simulink model "HIL_Testing_SW_amantest"  (Simulink 7.5)
settings: Solver=ode1  StartTime=0.0  StopTime=Inf  FixedStep=0.001  RelTol=1e-3
PostLoadFcn:
  | , if any(exist('dsrtsu_mdlpostloadfcn', 'file') == [2, 3, 6]), try dsrtsu_mdlpostloadfcn('Execute', bdroot); catch fprintf('Error in PostLoadFcn (dsrtsu_mdlpostloadfcn) for model "%s":\n %s\n', bdroot, lasterr); end, end,
undefined symbols (not defined in the file): CeBSER_Cnt_NumTempAxisPts, ChargeCord, ChargeCord_Control, ChargeToSOCCurr, ChrgCurrLim, CrntSens1Fine, CS_SOCSetPt, CyclerMaxChrgPwr, CyclerMaxDschrgPwr, deltaAhr, Drive_1, Drive_10, Drive_11, Drive_12, Drive_13, Drive_14, Drive_15, Drive_16, Drive_17, Drive_18, Drive_19, Drive_2, Drive_20, Drive_21, Drive_22, Drive_23, Drive_24, Drive_25, Drive_26, Drive_27, Drive_28, Drive_29, Drive_3, Drive_30, Drive_31, Drive_32, Drive_33, Drive_34, Drive_35, Drive_36, Drive_37, Drive_38, Drive_39, Drive_4, Drive_40, Drive_41, Drive_42, Drive_43, Drive_44, Drive_45, Drive_46, Drive_47, Drive_48, Drive_49, Drive_5, Drive_50, Drive_51, Drive_6, Drive_7, Drive_8 ... (+50)
libraries: simulink x129, rtican x50, rti2211sailib x5, rti2211serlib x5, rti2202miolib x3
(part 14 of 23)

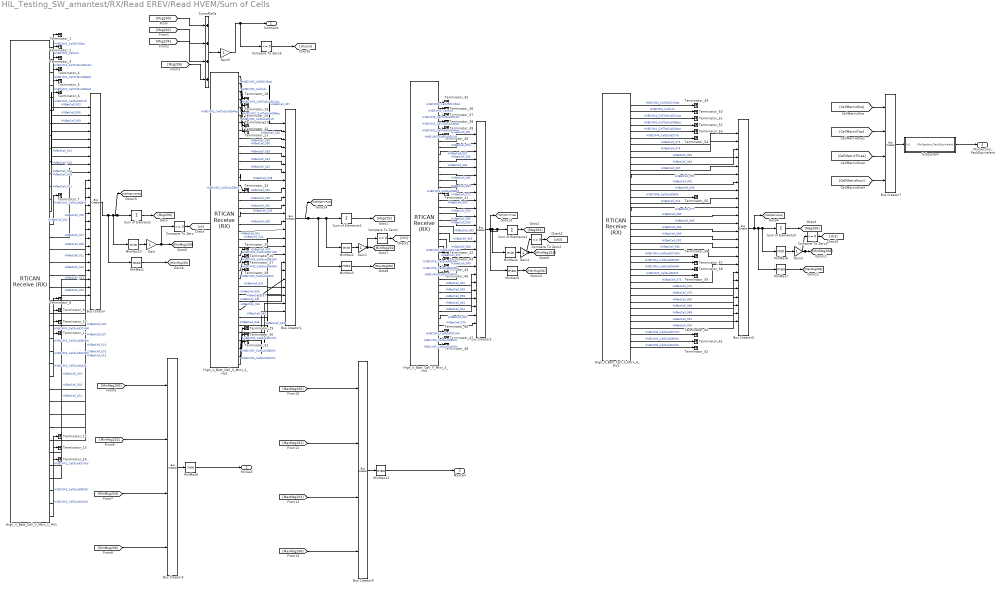
== system HIL_Testing_SW_amantest/RX/Read EREV/Read HVEM/Sum of Cells ==
  Bus Creator{,1..3} (4 alike) : BusCreator  Inputs=24
  Bus Creator5 : BusCreator
  Bus Creator6 : BusCreator
  Bus Creator7 : BusCreator
  Compare To Zero{,1..3,5} (5 alike) : simulink/Logic and Bit Operations/Compare To Zero  SystemSampleTime=-1  relop=<=  LogicOutDataTypeMode=uint8  ZeroCross=off
  Gain{,1..3,5} (5 alike) : Gain  ParameterDataType=sfix(16)  ParameterScaling=2^0  OutDataType=sfix(16)  OutScaling=2^0
  High_V_Batt_Cell_V_Mtrx_1_HV1 : rtican/RTICAN Receive (RX)   SystemSampleTime=-1  Reserved1=[]  Reserved2=[]  Reserved3=[]  Reserved4=[]  SfcnMessage=[]  Msg_Struct=[]  BoardTypeNo=[]  BoardNo=[]  ChannelNo=[]  Parameters=[]  DialogFcn=[]  UnitName=[]  Revision=[]  UnitValues=[]  DSProperties=struct('RTI',struct('Version',uint32(5),'BlockType',struct('isSLSource',uint8(1),'isSLSink',uint8(1),'isHWSource',uint8(0),'isHWSink',uint8(0),'isSetup',uint8(0),'isInline',uint8(1),'isNonInline',uint8(0),'isInterrupt',uint8(0),'isChannelwise',uint8(0)),'IOBoardType','RTICAN','UnitType','MESSAGE','Identifier','RX','DialogType','MSVC','BlockSet','RTICAN','SlaveProcessor','CAN'))  RTIBlockInterface=struct('OutputPortsWidth',int32([1 1 1 1 1 1 1 1 1 1 1 1 1 1 1 1 1 1 1 1 1 1 1 1 1 1 1 1 1 1 1 1 1 1 1 1 1 1]),'OutputPortsActive',[1 1 1 1 1 1 1 1 1 1 1 1 1 1 1 1 1 1 1 1 1 1 1 1 1 1 1 1 1 1 1 1 1 1 1 1 1 1],'OutputPortsName',{{'HVBCVM1_CellOCVStat','HVBCVM1_CellIndx','HVBCVM1_CellTstSubIDCAct','HVBCVM1_CellTstSubIDBAct','HVBCVM1_CellTstSubIDAAct','HVBCVM1_CellSubIDCVlt','HVBatCell_003','HVBatCell_006','HVBatCell_009','HVBatCell_012','HVBatCell_015','HVBatCell_018','HVBatCell_021','HVBatCell_024','HVBCVM1_CellSubIDBVlt','HVBatCell_002','HVBatCell_005','HVBatCell_008','HVBatCell_011','HVBatCell_014','HVBatCell_017','HVBatCell_020','HVBatCell_023','HVBCVM1_CellSubIDCVltM','HVBCVM1_CellSubIDBVltM','HVBCVM1_CellSubIDAVltM','HVBCVM1_CellSubIDAVlt','HVBatCell_001','HVBatCell_004','HVBatCell_007','HVBatCell_010','HVBatCell_013','HVBatCell_016','HVBatCell_019','HVBatCell_022','HVBCVM1_CellSubIDCVltV','HVBCVM1_CellSubIDBVltV','HVBCVM1_CellSubIDAVltV'}},'OutputPortsDataType',{{'SS_DOUBLE','SS_DOUBLE','SS_DOUBLE','SS_DOUBLE','SS_DOUBLE','SS_DOUBLE','SS_DOUBLE','SS_DOUBLE','SS_DOUBLE','SS_DOUBLE','SS_DOUBLE','SS_DOUBLE','SS_DOUBLE','SS_DOUBLE','SS_DOUBLE','SS_DOUBLE','SS_DOUBLE','SS_DOUBLE','SS_DOUBLE','SS_DOUBLE','SS_DOUBLE','SS_DOUBLE','SS_DOUBLE','SS_DOUBLE','SS_DOUBLE','SS_DOUBLE','SS_DOUBLE','SS_DOUBLE','SS_DOUBLE','SS_DOUBLE','SS_DOUBLE','SS_DOUBLE','SS_DOUBLE','SS_DOUBLE','SS_DOUBLE','SS_DOUBLE','SS_DOUBLE','SS_DOUBLE'}},'OutputPortsLabel',{{'HVBCVM1_CellOCVStat','HVBCVM1_CellIndx','HVBCVM1_CellTstSubIDCAct','HVBCVM1_CellTstSubIDBAct','HVBCVM1_CellTstSubIDAAct','HVBCVM1_CellSubIDCVlt','HVBatCell_003','HVBatCell_006','HVBatCell_009','HVBatCell_012','HVBatCell_015','HVBatCell_018','HVBatCell_021','HVBatCell_024','HVBCVM1_CellSubIDBVlt','HVBatCell_002','HVBatCell_005','HVBatCell_008','HVBatCell_011','HVBatCell_014','HVBatCell_017','HVBatCell_020','HVBatCell_023','HVBCVM1_CellSubIDCVltM','HVBCVM1_CellSubIDBVltM','HVBCVM1_CellSubIDAVltM','HVBCVM1_CellSubIDAVlt','HVBatCell_001','HVBatCell_004','HVBatCell_007','HVBatCell_010','HVBatCell_013','HVBatCell_016','HVBatCell_019','HVBatCell_022','HVBCVM1_CellSubIDCVltV','HVBCVM1_CellSubIDBVltV','HVBCVM1_CellSubIDAVltV'}},'OutputPortsLabelMode','ON','InputPortsWidth',int32(0),'InputPortsActive',0,'DialogFcn','rtican_message_interface_gui','BlockDisplay',{{'','center'}},'IconTransparency','on','ParameterTunableNames',{{}},'InitLevel',3,'BlockName',struct('Token',{{'High_V_Batt_Cell_V_Mtrx_1_HV'}}),'SampleTime',{{-1}},'TriggerPort',{{'none'}},'EnablePort',{{'none'}})  RTIBlockParameters=struct('BoardTypeNo',{{4302,'OFF',[]}},'BoardNo',{{1,'ON',[1 16]}},'ChannelNo',{{4,'ON',[1 4]}},'Parameters',{{struct('DataFileSupport',struct('DataFileSelectedMaster',1,'DataFileSelectedLocal',1,'DataFileName',['c:\data\databases\8.0.0 (12505)\globala - hv.dbc|c:\data\testing\dbc\globala - hvdmx112.dbc|'],'DataFileDate',{{{['06-Jan-2012 10:17:38']},{['10-May-2011 15:46:00']}}},'SelectedFile',['dbc\globala - hvdmx112.dbc']),'Options',struct('StatusSelected',0,'TimeSelected',0,'DeltaTimeSelected',0,'BytePortSelected',0,'MessageLengthSelected',0,'TriggerPort',struct('Selected',0,'TriggerType',0),'UserCoding',struct('Selected',0,'InterfaceFile','UserDecodingFile','FcnName','UserDecodeFcn','InportSelected',0,'InportWidth',1,'OutportSelected',0,'OutportWidth',1),'EnablePortSelected',0,'SignalOnPortnameSelected',1,'UseRXService',0),'Message',struct('MsgOnBlocknameSelected',1,'MsgName','High_V_Batt_Cell_V_Mtrx_1_HV','MsgIdFormat',0,'MsgId',512,'MsgLength',8,'NumSignals',38,'SampleTime',-1,'Signal',struct('SgnName',{'HVBCVM1_CellOCVStat','HVBCVM1_CellIndx','HVBCVM1_CellTstSubIDCAct','HVBCVM1_CellTstSubIDBAct','HVBCVM1_CellTstSubIDAAct','HVBCVM1_CellSubIDCVlt','HVBatCell_003','HVBatCell_006','HVBatCell_009','HVBatCell_012','HVBatCell_015','HVBatCell_018','HVBatCell_021','HVBatCell_024','HVBCVM1_CellSubIDBVlt','HVBatCell_002','HVBatCell_005','HVBatCell_008','HVBatCell_011','HVBatCell_014','HVBatCell_017','HVBatCell_020','HVBatCell_023','HVBCVM1_CellSubIDCVltM','HVBCVM1_CellSubIDBVltM','HVBCVM1_CellSubIDAVltM','HVBCVM1_CellSubIDAVlt','HVBatCell_001','HVBatCell_004','HVBatCell_007','HVBatCell_010','HVBatCell_013','HVBatCell_016','HVBatCell_019','HVBatCell_022','HVBCVM1_CellSubIDCVltV','HVBCVM1_CellSubIDBVltV','HVBCVM1_CellSubIDAVltV'},'SgnStartBit',{11,12,16,17,18,19,19,19,19,19,19,19,19,19,32,32,32,32,32,32,32,32,32,45,46,47,48,48,48,48,48,48,48,48,48,61,62,63},'SgnLength',{1,4,1,1,1,13,13,13,13,13,13,13,13,13,13,13,13,13,13,13,13,13,13,1,1,1,13,13,13,13,13,13,13,13,13,1,1,1},'SgnType',{0,1,0,0,0,0,2,2,2,2,2,2,2,2,0,2,2,2,2,2,2,2,2,0,0,0,0,2,2,2,2,2,2,2,2,0,0,0},'ModeValue',{-1,-1,-1,-1,-1,-1,1,3,5,7,9,11,13,15,-1,1,3,5,7,9,11,13,15,-1,-1,-1,-1,1,3,5,7,9,11,13,15,-1,-1,-1},'DataType',{0,0,0,0,0,0,0,0,0,0,0,0,0,0,0,0,0,0,0,0,0,0,0,0,0,0,0,0,0,0,0,0,0,0,0,0,0,0},'ByteLayout',{2,2,2,2,2,2,2,2,2,2,2,2,2,2,2,2,2,2,2,2,2,2,2,2,2,2,2,2,2,2,2,2,2,2,2,2,2,2},'Factor',{1,1,1,1,1,0.000625,0.000625,0.000625,0.000625,0.000625,0.000625,0.000625,0.000625,0.000625,0.000625,0.000625,0.000625,0.000625,0.000625,0.000625,0.000625,0.000625,0.000625,1,1,1,0.000625,0.000625,0.000625,0.000625,0.000625,0.000625,0.000625,0.000625,0.000625,1,1,1},'Offset',{0,0,0,0,0,0,0,0,0,0,0,0,0,0,0,0,0,0,0,0,0,0,0,0,0,0,0,0,0,0,0,0,0,0,0,0,0,0},'SgnComment',{{''},{''},{''},{''},{''},{''},{''},{''},{''},{''},{''},{''},{''},{''},{''},{''},{''},{''},{''},{''},{''},{''},{''},{''},{''},{''},{''},{''},{''},{''},{''},{''},{''},{''},{''},{''},{''},{''}},'SgnUnit',{'','','','','','V','V','V','V','V','V','V','V','V','V','V','V','V','V','V','V','V','V','','','','V','V','V','V','V','V','V','V','V','','',''},'Min',{0,0,0,0,0,0,0,0,0,0,0,0,0,0,0,0,0,0,0,0,0,0,0,0,0,0,0,0,0,0,0,0,0,0,0,0,0,0},'Max',{0,15,1,1,1,5.119375,5.119375,5.119375,5.119375,5.119375,5.119375,5.119375,5.119375,5.119375,5.119375,5.119375,5.119375,5.119375,5.119375,5.119375,5.119375,5.119375,5.119375,0,0,0,5.119375,5.119375,5.119375,5.119375,5.119375,5.119375,5.119375,5.119375,5.119375,0,0,0},'SLDataType',{'SS_DOUBLE','SS_DOUBLE','SS_DOUBLE','SS_DOUBLE','SS_DOUBLE','SS_DOUBLE','SS_DOUBLE','SS_DOUBLE','SS_DOUBLE','SS_DOUBLE','SS_DOUBLE','SS_DOUBLE','SS_DOUBLE','SS_DOUBLE','SS_DOUBLE','SS_DOUBLE','SS_DOUBLE','SS_DOUBLE','SS_DOUBLE','SS_DOUBLE','SS_DOUBLE','SS_DOUBLE','SS_DOUBLE','SS_DOUBLE','SS_DOUBLE','SS_DOUBLE','SS_DOUBLE','SS_DOUBLE','SS_DOUBLE','SS_DOUBLE','SS_DOUBLE','SS_DOUBLE','SS_DOUBLE','SS_DOUBLE','SS_DOUBLE','SS_DOUBLE','SS_DOUBLE','SS_DOUBLE'}),'MsgIdNumFormat',0,'MsgComment',{{''}}),'Version',1.2,'general',struct('isFromLib',0)),'OFF',[]}},'GroupId',{{struct('Group',{{'RTICAN'}},'No',7,'Behavior',{{'NAMECHANGE'}},'BlockType',{{'SINK'}},'NameChangeFlag',0),'OFF',[]}},'SFcnRTICANMessage',{{struct('MsgType','RX','SFcnPortType','Scalar','MsgName','High_V_Batt_Cell_V_Mtrx_1_HV','MsgIdFormat','STD','MsgId',512,'MsgLength',8,'NumSignals',38,'SampleTime',-1,'Signal',struct('SgnName',{'HVBCVM1_CellOCVStat','HVBCVM1_CellIndx','HVBCVM1_CellTstSubIDCAct','HVBCVM1_CellTstSubIDBAct','HVBCVM1_CellTstSubIDAAct','HVBCVM1_CellSubIDCVlt','HVBatCell_003','HVBatCell_006','HVBatCell_009','HVBatCell_012','HVBatCell_015','HVBatCell_018','HVBatCell_021','HVBatCell_024','HVBCVM1_CellSubIDBVlt','HVBatCell_002','HVBatCell_005','HVBatCell_008','HVBatCell_011','HVBatCell_014','HVBatCell_017','HVBatCell_020','HVBatCell_023','HVBCVM1_CellSubIDCVltM','HVBCVM1_CellSubIDBVltM','HVBCVM1_CellSubIDAVltM','HVBCVM1_CellSubIDAVlt','HVBatCell_001','HVBatCell_004','HVBatCell_007','HVBatCell_010','HVBatCell_013','HVBatCell_016','HVBatCell_019','HVBatCell_022','HVBCVM1_CellSubIDCVltV','HVBCVM1_CellSubIDBVltV','HVBCVM1_CellSubIDAVltV'},'SgnStartBit',{11,12,16,17,18,19,19,19,19,19,19,19,19,19,32,32,32,32,32,32,32,32,32,45,46,47,48,48,48,48,48,48,48,48,48,61,62,63},'SgnLength',{1,4,1,1,1,13,13,13,13,13,13,13,13,13,13,13,13,13,13,13,13,13,13,1,1,1,13,13,13,13,13,13,13,13,13,1,1,1},'SgnType',{'standard','mode','standard','standard','standard','standard','mode-dependent','mode-dependent','mode-dependent','mode-dependent','mode-dependent','mode-dependent','mode-dependent','mode-dependent','standard','mode-dependent','mode-dependent','mode-dependent','mode-dependent','mode-dependent','mode-dependent','mode-dependent','mode-dependent','standard','standard','standard','standard','mode-dependent','mode-dependent','mode-dependent','mode-dependent','mode-dependent','mode-dependent','mode-dependent','mode-dependent','standard','standard','standard'},'ModeValue',{-1,-1,-1,-1,-1,-1,1,3,5,7,9,11,13,15,-1,1,3,5,7,9,11,13,15,-1,-1,-1,-1,1,3,5,7,9,11,13,15,-1,-1,-1},'DataType',{['unsigned int'],['unsigned int'],['unsigned int'],['unsigned int'],['unsigned int'],['unsigned int'],['unsigned int'],['unsigned int'],['unsigned int'],['unsigned int'],['unsigned int'],['unsigned int'],['unsigned int'],['unsigned int'],['unsigned int'],['unsigned int'],['unsigned int'],['unsigned int'],['unsigned int'],['unsigned int'],['unsigned int'],['unsigned int'],['unsigned int'],['unsigned int'],['unsigned int'],['unsigned int'],['unsigned int'],['unsigned int'],['unsigned int'],['unsigned int'],['unsigned int'],['unsigned int'],['unsigned int'],['unsigned int'],['unsigned int'],['unsigned int'],['unsigned int'],['unsigned int']},'ByteLayout',{['motorola back.'],['motorola back.'],['motorola back.'],['motorola back.'],['motorola back.'],['motorola back.'],['motorola back.'],['motorola back.'],['motorola back.'],['motorola back.'],['motorola back.'],['motorola back.'],['motorola back.'],['motorola back.'],['motorola back.'],['motorola back.'],['motorola back.'],['motorola back.'],['motorola back.'],['motorola back.'],['motorola back.'],['motorola back.'],['motorola back.'],['motorola back.'],['motorola back.'],['motorola back.'],['motorola back.'],['motorola back.'],['motorola back.'],['motorola back.'],['motorola back.'],['motorola back.'],['motorola back.'],['motorola back.'],['motorola back.'],['motorola back.'],['motorola back.'],['motorola back.']},'Factor',{1,1,1,1,1,0.000625,0.000625,0.000625,0.000625,0.000625,0.000625,0.000625,0.000625,0.000625,0.000625,0.000625,0.000625,0.000625,0.000625,0.000625,0.000625,0.000625,0.000625,1,1,1,0.000625,0.000625,0.000625,0.000625,0.000625,0.000625,0.000625,0.000625,0.000625,1,1,1},'Offset',{0,0,0,0,0,0,0,0,0,0,0,0,0,0,0,0,0,0,0,0,0,0,0,0,0,0,0,0,0,0,0,0,0,0,0,0,0,0},'SLDataType',{'SS_DOUBLE','SS_DOUBLE','SS_DOUBLE','SS_DOUBLE','SS_DOUBLE','SS_DOUBLE','SS_DOUBLE','SS_DOUBLE','SS_DOUBLE','SS_DOUBLE','SS_DOUBLE','SS_DOUBLE','SS_DOUBLE','SS_DOUBLE','SS_DOUBLE','SS_DOUBLE','SS_DOUBLE','SS_DOUBLE','SS_DOUBLE','SS_DOUBLE','SS_DOUBLE','SS_DOUBLE','SS_DOUBLE','SS_DOUBLE','SS_DOUBLE','SS_DOUBLE','SS_DOUBLE','SS_DOUBLE','SS_DOUBLE','SS_DOUBLE','SS_DOUBLE','SS_DOUBLE','SS_DOUBLE','SS_DOUBLE','SS_DOUBLE','SS_DOUBLE','SS_DOUBLE','SS_DOUBLE'}),'StatusSelected','no','TimeSelected','no','DeltaTimeSelected','no','BytePortSelected','no','MessageLengthSelected','no','TriggerPort',struct('Selected','no','TriggerType',0),'UserCoding',struct('Selected','no','InterfaceFile','UserDecodingFile','FcnName','UserDecodeFcn','InportSelected','no','InportWidth',1,'OutportSelected','no','OutportWidth',1),'EnablePortSelected','no','UseRXService','no','BoardType','DS4302','BoardNo',1,'ControllerNo',4),'OFF',[]}},'TLCFileName',{{'rtican_rx_message','OFF',[]}})  RTISFcnParameters=struct('SFcnRTICANMessage','struct','TLCFileName','char')  RTIBlockParaDefault=struct('BoardTypeNo',4302,'BoardNo',1,'ChannelNo',1,'Parameters',struct('DataFileSupport',struct('DataFileSelectedMaster',0,'DataFileSelectedLocal',0,'DataFileName','','DataFileDate','','SelectedFile',['<no file selected>']),'Options',struct('StatusSelected',1,'TimeSelected',1,'DeltaTimeSelected',1,'BytePortSelected',0,'MessageLengthSelected',0,'TriggerPort',struct('Selected',0,'TriggerType','rising'),'UserCoding',struct('Selected',0,'InterfaceFile','UserDecodingFile','FcnName','UserDecodeFcn','InportSelected',0,'InportWidth',1,'OutportSelected',0,'OutportWidth',1),'EnablePortSelected',0,'SignalOnPortnameSelected',1,'UseRXService',0),'Message',struct('MsgOnBlocknameSelected',0,'MsgName',['RX Message'],'MsgIdFormat',0,'MsgId',100,'MsgLength',8,'NumSignals',1,'SampleTime',-1,'Signal',struct('SgnName',['RX signal'],'SgnStartBit',0,'SgnLength',8,'SgnType',0,'ModeValue',-1,'DataType',0,'SLDataType','SS_DOUBLE','ByteLayout',0,'Factor',1,'Offset',0,'Min',0,'Max',255,'SgnComment',{{}},'SgnUnit',''),'MsgIdNumFormat',0,'MsgComment',{{''}}),'Version',1.2,'general',struct('isFromLib',1)),'GroupId',struct('Group',{{'RTICAN'}},'No',1,'Behavior',{{'NAMECHANGE'}},'BlockType',{{'SINK'}},'NameChangeFlag',0),'SFcnRTICANMessage',struct('MsgType','RX','MsgName',['RX Message'],'MsgIdFormat','STD','MsgId',100,'MsgLength',8,'NumSignals',1,'SampleTime',-1,'Signal',struct('SgnName',['RX signal'],'SgnStartBit',0,'SgnLength',8,'SgnType','standard','ModeValue',-1,'DataType',['unsigned int'],'ByteLayout',['little endian'],'SLDataType','SS_DOUBLE','Factor',1,'Offset',0),'StatusSelected','yes','TimeSelected','yes','DeltaTimeSelected','yes','BytePortSelected','no','MessageLengthSelected','no','EnablePortSelected','no','UserCoding',struct('Selected','no','InterfaceFile','UserDecodingFile','FcnName','UserDecodeFcn','InportSelected','no','InportWidth',1,'OutportSelected','no','OutportWidth',1),'TriggerPort',struct('Selected','no','TriggerType','rising'),'UseRXService','no','BoardType','DS4302','BoardNo',1,'ControllerNo',1,'SFcnPortType','Scalar'),'TLCFileName','rtican_rx_message')
      settings: AttributesFormatString=Group Id: RTICAN7\n
  High_V_Batt_Cell_V_Mtrx_2_HV1 : rtican/RTICAN Receive (RX)   SystemSampleTime=-1  Reserved1=[]  Reserved2=[]  Reserved3=[]  Reserved4=[]  SfcnMessage=[]  Msg_Struct=[]  BoardTypeNo=[]  BoardNo=[]  ChannelNo=[]  Parameters=[]  DialogFcn=[]  UnitName=[]  Revision=[]  UnitValues=[]  DSProperties=struct('RTI',struct('Version',uint32(5),'BlockType',struct('isSLSource',uint8(1),'isSLSink',uint8(1),'isHWSource',uint8(0),'isHWSink',uint8(0),'isSetup',uint8(0),'isInline',uint8(1),'isNonInline',uint8(0),'isInterrupt',uint8(0),'isChannelwise',uint8(0)),'IOBoardType','RTICAN','UnitType','MESSAGE','Identifier','RX','DialogType','MSVC','BlockSet','RTICAN','SlaveProcessor','CAN'))  RTIBlockInterface=struct('OutputPortsWidth',int32([1 1 1 1 1 1 1 1 1 1 1 1 1 1 1 1 1 1 1 1 1 1 1 1 1 1 1 1 1 1 1 1 1 1 1 1 1 1]),'OutputPortsActive',[1 1 1 1 1 1 1 1 1 1 1 1 1 1 1 1 1 1 1 1 1 1 1 1 1 1 1 1 1 1 1 1 1 1 1 1 1 1],'OutputPortsName',{{'HVBCVM2_CellOCVStat','HVBCVM2_CellIndx','HVBCVM2_CellTstSubIDCAct','HVBCVM2_CellTstSubIDBAct','HVBCVM2_CellTstSubIDAAct','HVBCVM2_CellSubIDCVlt','HVBatCell_027','HVBatCell_030','HVBatCell_033','HVBatCell_036','HVBatCell_039','HVBatCell_042','HVBatCell_045','HVBatCell_048','HVBCVM2_CellSubIDBVlt','HVBatCell_026','HVBatCell_029','HVBatCell_032','HVBatCell_035','HVBatCell_038','HVBatCell_041','HVBatCell_044','HVBatCell_047','HVBCVM2_CellSubIDCVltM','HVBCVM2_CellSubIDBVltM','HVBCVM2_CellSubIDAVltM','HVBCVM2_CellSubIDAVlt','HVBatCell_025','HVBatCell_028','HVBatCell_031','HVBatCell_034','HVBatCell_037','HVBatCell_040','HVBatCell_043','HVBatCell_046','HVBCVM2_CellSubIDCVltV','HVBCVM2_CellSubIDBVltV','HVBCVM2_CellSubIDAVltV'}},'OutputPortsDataType',{{'SS_DOUBLE','SS_DOUBLE','SS_DOUBLE','SS_DOUBLE','SS_DOUBLE','SS_DOUBLE','SS_DOUBLE','SS_DOUBLE','SS_DOUBLE','SS_DOUBLE','SS_DOUBLE','SS_DOUBLE','SS_DOUBLE','SS_DOUBLE','SS_DOUBLE','SS_DOUBLE','SS_DOUBLE','SS_DOUBLE','SS_DOUBLE','SS_DOUBLE','SS_DOUBLE','SS_DOUBLE','SS_DOUBLE','SS_DOUBLE','SS_DOUBLE','SS_DOUBLE','SS_DOUBLE','SS_DOUBLE','SS_DOUBLE','SS_DOUBLE','SS_DOUBLE','SS_DOUBLE','SS_DOUBLE','SS_DOUBLE','SS_DOUBLE','SS_DOUBLE','SS_DOUBLE','SS_DOUBLE'}},'OutputPortsLabel',{{'HVBCVM2_CellOCVStat','HVBCVM2_CellIndx','HVBCVM2_CellTstSubIDCAct','HVBCVM2_CellTstSubIDBAct','HVBCVM2_CellTstSubIDAAct','HVBCVM2_CellSubIDCVlt','HVBatCell_027','HVBatCell_030','HVBatCell_033','HVBatCell_036','HVBatCell_039','HVBatCell_042','HVBatCell_045','HVBatCell_048','HVBCVM2_CellSubIDBVlt','HVBatCell_026','HVBatCell_029','HVBatCell_032','HVBatCell_035','HVBatCell_038','HVBatCell_041','HVBatCell_044','HVBatCell_047','HVBCVM2_CellSubIDCVltM','HVBCVM2_CellSubIDBVltM','HVBCVM2_CellSubIDAVltM','HVBCVM2_CellSubIDAVlt','HVBatCell_025','HVBatCell_028','HVBatCell_031','HVBatCell_034','HVBatCell_037','HVBatCell_040','HVBatCell_043','HVBatCell_046','HVBCVM2_CellSubIDCVltV','HVBCVM2_CellSubIDBVltV','HVBCVM2_CellSubIDAVltV'}},'OutputPortsLabelMode','ON','InputPortsWidth',int32(0),'InputPortsActive',0,'DialogFcn','rtican_message_interface_gui','BlockDisplay',{{'','center'}},'IconTransparency','on','ParameterTunableNames',{{}},'InitLevel',3,'BlockName',struct('Token',{{'High_V_Batt_Cell_V_Mtrx_2_HV'}}),'SampleTime',{{-1}},'TriggerPort',{{'none'}},'EnablePort',{{'none'}})  RTIBlockParameters=struct('BoardTypeNo',{{4302,'OFF',[]}},'BoardNo',{{1,'ON',[1 16]}},'ChannelNo',{{4,'ON',[1 4]}},'Parameters',{{struct('DataFileSupport',struct('DataFileSelectedMaster',1,'DataFileSelectedLocal',1,'DataFileName',['c:\data\databases\6.4.1\globala - hv.dbc|c:\data\testing\dbc\globala - hvdmx112.dbc|'],'DataFileDate',{{{['06-Jan-2012 10:17:38']},{['10-May-2011 15:46:00']}}},'SelectedFile',['dbc\globala - hvdmx112.dbc']),'Options',struct('StatusSelected',0,'TimeSelected',0,'DeltaTimeSelected',0,'BytePortSelected',0,'MessageLengthSelected',0,'TriggerPort',struct('Selected',0,'TriggerType',0),'UserCoding',struct('Selected',0,'InterfaceFile','UserDecodingFile','FcnName','UserDecodeFcn','InportSelected',0,'InportWidth',1,'OutportSelected',0,'OutportWidth',1),'EnablePortSelected',0,'SignalOnPortnameSelected',1,'UseRXService',0),'Message',struct('MsgOnBlocknameSelected',1,'MsgName','High_V_Batt_Cell_V_Mtrx_2_HV','MsgIdFormat',0,'MsgId',514,'MsgLength',8,'NumSignals',38,'SampleTime',-1,'Signal',struct('SgnName',{'HVBCVM2_CellOCVStat','HVBCVM2_CellIndx','HVBCVM2_CellTstSubIDCAct','HVBCVM2_CellTstSubIDBAct','HVBCVM2_CellTstSubIDAAct','HVBCVM2_CellSubIDCVlt','HVBatCell_027','HVBatCell_030','HVBatCell_033','HVBatCell_036','HVBatCell_039','HVBatCell_042','HVBatCell_045','HVBatCell_048','HVBCVM2_CellSubIDBVlt','HVBatCell_026','HVBatCell_029','HVBatCell_032','HVBatCell_035','HVBatCell_038','HVBatCell_041','HVBatCell_044','HVBatCell_047','HVBCVM2_CellSubIDCVltM','HVBCVM2_CellSubIDBVltM','HVBCVM2_CellSubIDAVltM','HVBCVM2_CellSubIDAVlt','HVBatCell_025','HVBatCell_028','HVBatCell_031','HVBatCell_034','HVBatCell_037','HVBatCell_040','HVBatCell_043','HVBatCell_046','HVBCVM2_CellSubIDCVltV','HVBCVM2_CellSubIDBVltV','HVBCVM2_CellSubIDAVltV'},'SgnStartBit',{11,12,16,17,18,19,19,19,19,19,19,19,19,19,32,32,32,32,32,32,32,32,32,45,46,47,48,48,48,48,48,48,48,48,48,61,62,63},'SgnLength',{1,4,1,1,1,13,13,13,13,13,13,13,13,13,13,13,13,13,13,13,13,13,13,1,1,1,13,13,13,13,13,13,13,13,13,1,1,1},'SgnType',{0,1,0,0,0,2,2,2,2,2,2,2,2,2,2,2,2,2,2,2,2,2,2,0,0,0,2,2,2,2,2,2,2,2,2,0,0,0},'ModeValue',{-1,-1,-1,-1,-1,1,1,3,5,7,9,11,13,15,1,1,3,5,7,9,11,13,15,-1,-1,-1,1,1,3,5,7,9,11,13,15,-1,-1,-1},'DataType',{0,0,0,0,0,0,0,0,0,0,0,0,0,0,0,0,0,0,0,0,0,0,0,0,0,0,0,0,0,0,0,0,0,0,0,0,0,0},'ByteLayout',{2,2,2,2,2,2,2,2,2,2,2,2,2,2,2,2,2,2,2,2,2,2,2,2,2,2,2,2,2,2,2,2,2,2,2,2,2,2},'Factor',{1,1,1,1,1,0.000625,0.000625,0.000625,0.000625,0.000625,0.000625,0.000625,0.000625,0.000625,0.000625,0.000625,0.000625,0.000625,0.000625,0.000625,0.000625,0.000625,0.000625,1,1,1,0.000625,0.000625,0.000625,0.000625,0.000625,0.000625,0.000625,0.000625,0.000625,1,1,1},'Offset',{0,0,0,0,0,0,0,0,0,0,0,0,0,0,0,0,0,0,0,0,0,0,0,0,0,0,0,0,0,0,0,0,0,0,0,0,0,0},'SgnComment',{{''},{''},{''},{''},{''},{''},{''},{''},{''},{''},{''},{''},{''},{''},{''},{''},{''},{''},{''},{''},{''},{''},{''},{''},{''},{''},{''},{''},{''},{''},{''},{''},{''},{''},{''},{''},{''},{''}},'SgnUnit',{'','','','','','V','V','V','V','V','V','V','V','V','V','V','V','V','V','V','V','V','V','','','','V','V','V','V','V','V','V','V','V','','',''},'Min',{0,0,0,0,0,0,0,0,0,0,0,0,0,0,0,0,0,0,0,0,0,0,0,0,0,0,0,0,0,0,0,0,0,0,0,0,0,0},'Max',{0,15,1,1,1,5.119375,5.119375,5.119375,5.119375,5.119375,5.119375,5.119375,5.119375,5.119375,5.119375,5.119375,5.119375,5.119375,5.119375,5.119375,5.119375,5.119375,5.119375,0,0,0,5.119375,5.119375,5.119375,5.119375,5.119375,5.119375,5.119375,5.119375,5.119375,0,0,0},'SLDataType',{'SS_DOUBLE','SS_DOUBLE','SS_DOUBLE','SS_DOUBLE','SS_DOUBLE','SS_DOUBLE','SS_DOUBLE','SS_DOUBLE','SS_DOUBLE','SS_DOUBLE','SS_DOUBLE','SS_DOUBLE','SS_DOUBLE','SS_DOUBLE','SS_DOUBLE','SS_DOUBLE','SS_DOUBLE','SS_DOUBLE','SS_DOUBLE','SS_DOUBLE','SS_DOUBLE','SS_DOUBLE','SS_DOUBLE','SS_DOUBLE','SS_DOUBLE','SS_DOUBLE','SS_DOUBLE','SS_DOUBLE','SS_DOUBLE','SS_DOUBLE','SS_DOUBLE','SS_DOUBLE','SS_DOUBLE','SS_DOUBLE','SS_DOUBLE','SS_DOUBLE','SS_DOUBLE','SS_DOUBLE'}),'MsgIdNumFormat',0,'MsgComment',{{''}}),'Version',1.2,'general',struct('isFromLib',0)),'OFF',[]}},'GroupId',{{struct('Group',{{'RTICAN'}},'No',7,'Behavior',{{'NAMECHANGE'}},'BlockType',{{'SINK'}},'NameChangeFlag',0),'OFF',[]}},'SFcnRTICANMessage',{{struct('MsgType','RX','SFcnPortType','Scalar','MsgName','High_V_Batt_Cell_V_Mtrx_2_HV','MsgIdFormat','STD','MsgId',514,'MsgLength',8,'NumSignals',38,'SampleTime',-1,'Signal',struct('SgnName',{'HVBCVM2_CellOCVStat','HVBCVM2_CellIndx','HVBCVM2_CellTstSubIDCAct','HVBCVM2_CellTstSubIDBAct','HVBCVM2_CellTstSubIDAAct','HVBCVM2_CellSubIDCVlt','HVBatCell_027','HVBatCell_030','HVBatCell_033','HVBatCell_036','HVBatCell_039','HVBatCell_042','HVBatCell_045','HVBatCell_048','HVBCVM2_CellSubIDBVlt','HVBatCell_026','HVBatCell_029','HVBatCell_032','HVBatCell_035','HVBatCell_038','HVBatCell_041','HVBatCell_044','HVBatCell_047','HVBCVM2_CellSubIDCVltM','HVBCVM2_CellSubIDBVltM','HVBCVM2_CellSubIDAVltM','HVBCVM2_CellSubIDAVlt','HVBatCell_025','HVBatCell_028','HVBatCell_031','HVBatCell_034','HVBatCell_037','HVBatCell_040','HVBatCell_043','HVBatCell_046','HVBCVM2_CellSubIDCVltV','HVBCVM2_CellSubIDBVltV','HVBCVM2_CellSubIDAVltV'},'SgnStartBit',{11,12,16,17,18,19,19,19,19,19,19,19,19,19,32,32,32,32,32,32,32,32,32,45,46,47,48,48,48,48,48,48,48,48,48,61,62,63},'SgnLength',{1,4,1,1,1,13,13,13,13,13,13,13,13,13,13,13,13,13,13,13,13,13,13,1,1,1,13,13,13,13,13,13,13,13,13,1,1,1},'SgnType',{'standard','mode','standard','standard','standard','mode-dependent','mode-dependent','mode-dependent','mode-dependent','mode-dependent','mode-dependent','mode-dependent','mode-dependent','mode-dependent','mode-dependent','mode-dependent','mode-dependent','mode-dependent','mode-dependent','mode-dependent','mode-dependent','mode-dependent','mode-dependent','standard','standard','standard','mode-dependent','mode-dependent','mode-dependent','mode-dependent','mode-dependent','mode-dependent','mode-dependent','mode-dependent','mode-dependent','standard','standard','standard'},'ModeValue',{-1,-1,-1,-1,-1,1,1,3,5,7,9,11,13,15,1,1,3,5,7,9,11,13,15,-1,-1,-1,1,1,3,5,7,9,11,13,15,-1,-1,-1},'DataType',{['unsigned int'],['unsigned int'],['unsigned int'],['unsigned int'],['unsigned int'],['unsigned int'],['unsigned int'],['unsigned int'],['unsigned int'],['unsigned int'],['unsigned int'],['unsigned int'],['unsigned int'],['unsigned int'],['unsigned int'],['unsigned int'],['unsigned int'],['unsigned int'],['unsigned int'],['unsigned int'],['unsigned int'],['unsigned int'],['unsigned int'],['unsigned int'],['unsigned int'],['unsigned int'],['unsigned int'],['unsigned int'],['unsigned int'],['unsigned int'],['unsigned int'],['unsigned int'],['unsigned int'],['unsigned int'],['unsigned int'],['unsigned int'],['unsigned int'],['unsigned int']},'ByteLayout',{['motorola back.'],['motorola back.'],['motorola back.'],['motorola back.'],['motorola back.'],['motorola back.'],['motorola back.'],['motorola back.'],['motorola back.'],['motorola back.'],['motorola back.'],['motorola back.'],['motorola back.'],['motorola back.'],['motorola back.'],['motorola back.'],['motorola back.'],['motorola back.'],['motorola back.'],['motorola back.'],['motorola back.'],['motorola back.'],['motorola back.'],['motorola back.'],['motorola back.'],['motorola back.'],['motorola back.'],['motorola back.'],['motorola back.'],['motorola back.'],['motorola back.'],['motorola back.'],['motorola back.'],['motorola back.'],['motorola back.'],['motorola back.'],['motorola back.'],['motorola back.']},'Factor',{1,1,1,1,1,0.000625,0.000625,0.000625,0.000625,0.000625,0.000625,0.000625,0.000625,0.000625,0.000625,0.000625,0.000625,0.000625,0.000625,0.000625,0.000625,0.000625,0.000625,1,1,1,0.000625,0.000625,0.000625,0.000625,0.000625,0.000625,0.000625,0.000625,0.000625,1,1,1},'Offset',{0,0,0,0,0,0,0,0,0,0,0,0,0,0,0,0,0,0,0,0,0,0,0,0,0,0,0,0,0,0,0,0,0,0,0,0,0,0},'SLDataType',{'SS_DOUBLE','SS_DOUBLE','SS_DOUBLE','SS_DOUBLE','SS_DOUBLE','SS_DOUBLE','SS_DOUBLE','SS_DOUBLE','SS_DOUBLE','SS_DOUBLE','SS_DOUBLE','SS_DOUBLE','SS_DOUBLE','SS_DOUBLE','SS_DOUBLE','SS_DOUBLE','SS_DOUBLE','SS_DOUBLE','SS_DOUBLE','SS_DOUBLE','SS_DOUBLE','SS_DOUBLE','SS_DOUBLE','SS_DOUBLE','SS_DOUBLE','SS_DOUBLE','SS_DOUBLE','SS_DOUBLE','SS_DOUBLE','SS_DOUBLE','SS_DOUBLE','SS_DOUBLE','SS_DOUBLE','SS_DOUBLE','SS_DOUBLE','SS_DOUBLE','SS_DOUBLE','SS_DOUBLE'}),'StatusSelected','no','TimeSelected','no','DeltaTimeSelected','no','BytePortSelected','no','MessageLengthSelected','no','TriggerPort',struct('Selected','no','TriggerType',0),'UserCoding',struct('Selected','no','InterfaceFile','UserDecodingFile','FcnName','UserDecodeFcn','InportSelected','no','InportWidth',1,'OutportSelected','no','OutportWidth',1),'EnablePortSelected','no','UseRXService','no','BoardType','DS4302','BoardNo',1,'ControllerNo',4),'OFF',[]}},'TLCFileName',{{'rtican_rx_message','OFF',[]}})  RTISFcnParameters=struct('SFcnRTICANMessage','struct','TLCFileName','char')  RTIBlockParaDefault=struct('BoardTypeNo',4302,'BoardNo',1,'ChannelNo',1,'Parameters',struct('DataFileSupport',struct('DataFileSelectedMaster',0,'DataFileSelectedLocal',0,'DataFileName','','DataFileDate','','SelectedFile',['<no file selected>']),'Options',struct('StatusSelected',1,'TimeSelected',1,'DeltaTimeSelected',1,'BytePortSelected',0,'MessageLengthSelected',0,'TriggerPort',struct('Selected',0,'TriggerType','rising'),'UserCoding',struct('Selected',0,'InterfaceFile','UserDecodingFile','FcnName','UserDecodeFcn','InportSelected',0,'InportWidth',1,'OutportSelected',0,'OutportWidth',1),'EnablePortSelected',0,'SignalOnPortnameSelected',1,'UseRXService',0),'Message',struct('MsgOnBlocknameSelected',0,'MsgName',['RX Message'],'MsgIdFormat',0,'MsgId',100,'MsgLength',8,'NumSignals',1,'SampleTime',-1,'Signal',struct('SgnName',['RX signal'],'SgnStartBit',0,'SgnLength',8,'SgnType',0,'ModeValue',-1,'DataType',0,'SLDataType','SS_DOUBLE','ByteLayout',0,'Factor',1,'Offset',0,'Min',0,'Max',255,'SgnComment',{{}},'SgnUnit',''),'MsgIdNumFormat',0,'MsgComment',{{''}}),'Version',1.2,'general',struct('isFromLib',1)),'GroupId',struct('Group',{{'RTICAN'}},'No',1,'Behavior',{{'NAMECHANGE'}},'BlockType',{{'SINK'}},'NameChangeFlag',0),'SFcnRTICANMessage',struct('MsgType','RX','MsgName',['RX Message'],'MsgIdFormat','STD','MsgId',100,'MsgLength',8,'NumSignals',1,'SampleTime',-1,'Signal',struct('SgnName',['RX signal'],'SgnStartBit',0,'SgnLength',8,'SgnType','standard','ModeValue',-1,'DataType',['unsigned int'],'ByteLayout',['little endian'],'SLDataType','SS_DOUBLE','Factor',1,'Offset',0),'StatusSelected','yes','TimeSelected','yes','DeltaTimeSelected','yes','BytePortSelected','no','MessageLengthSelected','no','EnablePortSelected','no','UserCoding',struct('Selected','no','InterfaceFile','UserDecodingFile','FcnName','UserDecodeFcn','InportSelected','no','InportWidth',1,'OutportSelected','no','OutportWidth',1),'TriggerPort',struct('Selected','no','TriggerType','rising'),'UseRXService','no','BoardType','DS4302','BoardNo',1,'ControllerNo',1,'SFcnPortType','Scalar'),'TLCFileName','rtican_rx_message')
      settings: AttributesFormatString=Group Id: RTICAN7\n
  High_V_Batt_Cell_V_Mtrx_3_HV1 : rtican/RTICAN Receive (RX)   SystemSampleTime=-1  Reserved1=[]  Reserved2=[]  Reserved3=[]  Reserved4=[]  SfcnMessage=[]  Msg_Struct=[]  BoardTypeNo=[]  BoardNo=[]  ChannelNo=[]  Parameters=[]  DialogFcn=[]  UnitName=[]  Revision=[]  UnitValues=[]  DSProperties=struct('RTI',struct('Version',uint32(5),'BlockType',struct('isSLSource',uint8(1),'isSLSink',uint8(1),'isHWSource',uint8(0),'isHWSink',uint8(0),'isSetup',uint8(0),'isInline',uint8(1),'isNonInline',uint8(0),'isInterrupt',uint8(0),'isChannelwise',uint8(0)),'IOBoardType','RTICAN','UnitType','MESSAGE','Identifier','RX','DialogType','MSVC','BlockSet','RTICAN','SlaveProcessor','CAN'))  RTIBlockInterface=struct('OutputPortsWidth',int32([1 1 1 1 1 1 1 1 1 1 1 1 1 1 1 1 1 1 1 1 1 1 1 1 1 1 1 1 1 1 1 1 1 1 1 1 1 1]),'OutputPortsActive',[1 1 1 1 1 1 1 1 1 1 1 1 1 1 1 1 1 1 1 1 1 1 1 1 1 1 1 1 1 1 1 1 1 1 1 1 1 1],'OutputPortsName',{{'HVBCVM3_CellVltOCVStat','HVBCVM3_CellIndx','HVBCVM3_CellTstSubIDCAct','HVBCVM3_CellTstSubIDBAct','HVBCVM3_CellTstSubIDAAct','HVBCVM3_CellSubIDCVlt','HVBatCell_051','HVBatCell_054','HVBatCell_057','HVBatCell_060','HVBatCell_063','HVBatCell_066','HVBatCell_069','HVBatCell_072','HVBCVM3_CellSubIDBVlt','HVBatCell_050','HVBatCell_053','HVBatCell_056','HVBatCell_059','HVBatCell_062','HVBatCell_065','HVBatCell_068','HVBatCell_071','HVBCVM3_CellSubIDCVltM','HVBCVM3_CellSubIDBVltM','HVBCVM3_CellSubIDAVltM','HVBCVM3_CellSubIDAVlt','HVBatCell_049','HVBatCell_052','HVBatCell_055','HVBatCell_058','HVBatCell_061','HVBatCell_064','HVBatCell_067','HVBatCell_070','HVBCVM3_CellSubIDCVltV','HVBCVM3_CellSubIDBVltV','HVBCVM3_CellSubIDAVltV'}},'OutputPortsDataType',{{'SS_DOUBLE','SS_DOUBLE','SS_DOUBLE','SS_DOUBLE','SS_DOUBLE','SS_DOUBLE','SS_DOUBLE','SS_DOUBLE','SS_DOUBLE','SS_DOUBLE','SS_DOUBLE','SS_DOUBLE','SS_DOUBLE','SS_DOUBLE','SS_DOUBLE','SS_DOUBLE','SS_DOUBLE','SS_DOUBLE','SS_DOUBLE','SS_DOUBLE','SS_DOUBLE','SS_DOUBLE','SS_DOUBLE','SS_DOUBLE','SS_DOUBLE','SS_DOUBLE','SS_DOUBLE','SS_DOUBLE','SS_DOUBLE','SS_DOUBLE','SS_DOUBLE','SS_DOUBLE','SS_DOUBLE','SS_DOUBLE','SS_DOUBLE','SS_DOUBLE','SS_DOUBLE','SS_DOUBLE'}},'OutputPortsLabel',{{'HVBCVM3_CellVltOCVStat','HVBCVM3_CellIndx','HVBCVM3_CellTstSubIDCAct','HVBCVM3_CellTstSubIDBAct','HVBCVM3_CellTstSubIDAAct','HVBCVM3_CellSubIDCVlt','HVBatCell_051','HVBatCell_054','HVBatCell_057','HVBatCell_060','HVBatCell_063','HVBatCell_066','HVBatCell_069','HVBatCell_072','HVBCVM3_CellSubIDBVlt','HVBatCell_050','HVBatCell_053','HVBatCell_056','HVBatCell_059','HVBatCell_062','HVBatCell_065','HVBatCell_068','HVBatCell_071','HVBCVM3_CellSubIDCVltM','HVBCVM3_CellSubIDBVltM','HVBCVM3_CellSubIDAVltM','HVBCVM3_CellSubIDAVlt','HVBatCell_049','HVBatCell_052','HVBatCell_055','HVBatCell_058','HVBatCell_061','HVBatCell_064','HVBatCell_067','HVBatCell_070','HVBCVM3_CellSubIDCVltV','HVBCVM3_CellSubIDBVltV','HVBCVM3_CellSubIDAVltV'}},'OutputPortsLabelMode','ON','InputPortsWidth',int32(0),'InputPortsActive',0,'DialogFcn','rtican_message_interface_gui','BlockDisplay',{{'','center'}},'IconTransparency','on','ParameterTunableNames',{{}},'InitLevel',3,'BlockName',struct('Token',{{'High_V_Batt_Cell_V_Mtrx_3_HV'}}),'SampleTime',{{-1}},'TriggerPort',{{'none'}},'EnablePort',{{'none'}})  RTIBlockParameters=struct('BoardTypeNo',{{4302,'OFF',[]}},'BoardNo',{{1,'ON',[1 16]}},'ChannelNo',{{4,'ON',[1 4]}},'Parameters',{{struct('DataFileSupport',struct('DataFileSelectedMaster',1,'DataFileSelectedLocal',1,'DataFileName',['c:\data\databases\6.4.1\globala - hv.dbc|c:\data\testing\dbc\globala - hvdmx112.dbc|'],'DataFileDate',{{{['06-Jan-2012 10:17:38']},{['10-May-2011 15:46:00']}}},'SelectedFile',['dbc\globala - hvdmx112.dbc']),'Options',struct('StatusSelected',0,'TimeSelected',0,'DeltaTimeSelected',0,'BytePortSelected',0,'MessageLengthSelected',0,'TriggerPort',struct('Selected',0,'TriggerType',0),'UserCoding',struct('Selected',0,'InterfaceFile','UserDecodingFile','FcnName','UserDecodeFcn','InportSelected',0,'InportWidth',1,'OutportSelected',0,'OutportWidth',1),'EnablePortSelected',0,'SignalOnPortnameSelected',1,'UseRXService',0),'Message',struct('MsgOnBlocknameSelected',1,'MsgName','High_V_Batt_Cell_V_Mtrx_3_HV','MsgIdFormat',0,'MsgId',516,'MsgLength',8,'NumSignals',38,'SampleTime',-1,'Signal',struct('SgnName',{'HVBCVM3_CellVltOCVStat','HVBCVM3_CellIndx','HVBCVM3_CellTstSubIDCAct','HVBCVM3_CellTstSubIDBAct','HVBCVM3_CellTstSubIDAAct','HVBCVM3_CellSubIDCVlt','HVBatCell_051','HVBatCell_054','HVBatCell_057','HVBatCell_060','HVBatCell_063','HVBatCell_066','HVBatCell_069','HVBatCell_072','HVBCVM3_CellSubIDBVlt','HVBatCell_050','HVBatCell_053','HVBatCell_056','HVBatCell_059','HVBatCell_062','HVBatCell_065','HVBatCell_068','HVBatCell_071','HVBCVM3_CellSubIDCVltM','HVBCVM3_CellSubIDBVltM','HVBCVM3_CellSubIDAVltM','HVBCVM3_CellSubIDAVlt','HVBatCell_049','HVBatCell_052','HVBatCell_055','HVBatCell_058','HVBatCell_061','HVBatCell_064','HVBatCell_067','HVBatCell_070','HVBCVM3_CellSubIDCVltV','HVBCVM3_CellSubIDBVltV','HVBCVM3_CellSubIDAVltV'},'SgnStartBit',{11,12,16,17,18,19,19,19,19,19,19,19,19,19,32,32,32,32,32,32,32,32,32,45,46,47,48,48,48,48,48,48,48,48,48,61,62,63},'SgnLength',{1,4,1,1,1,13,13,13,13,13,13,13,13,13,13,13,13,13,13,13,13,13,13,1,1,1,13,13,13,13,13,13,13,13,13,1,1,1},'SgnType',{0,1,0,0,0,2,2,2,2,2,2,2,2,2,2,2,2,2,2,2,2,2,2,0,0,0,2,2,2,2,2,2,2,2,2,0,0,0},'ModeValue',{-1,-1,-1,-1,-1,0,1,3,5,7,9,11,13,15,0,1,3,5,7,9,11,13,15,-1,-1,-1,0,1,3,5,7,9,11,13,15,-1,-1,-1},'DataType',{0,0,0,0,0,0,0,0,0,0,0,0,0,0,0,0,0,0,0,0,0,0,0,0,0,0,0,0,0,0,0,0,0,0,0,0,0,0},'ByteLayout',{2,2,2,2,2,2,2,2,2,2,2,2,2,2,2,2,2,2,2,2,2,2,2,2,2,2,2,2,2,2,2,2,2,2,2,2,2,2},'Factor',{1,1,1,1,1,0.000625,0.000625,0.000625,0.000625,0.000625,0.000625,0.000625,0.000625,0.000625,0.000625,0.000625,0.000625,0.000625,0.000625,0.000625,0.000625,0.000625,0.000625,1,1,1,0.000625,0.000625,0.000625,0.000625,0.000625,0.000625,0.000625,0.000625,0.000625,1,1,1},'Offset',{0,0,0,0,0,0,0,0,0,0,0,0,0,0,0,0,0,0,0,0,0,0,0,0,0,0,0,0,0,0,0,0,0,0,0,0,0,0},'SgnComment',{{''},{''},{''},{''},{''},{''},{''},{''},{''},{''},{''},{''},{''},{''},{''},{''},{''},{''},{''},{''},{''},{''},{''},{''},{''},{''},{''},{''},{''},{''},{''},{''},{''},{''},{''},{''},{''},{''}},'SgnUnit',{'','','','','','V','V','V','V','V','V','V','V','V','V','V','V','V','V','V','V','V','V','','','','V','V','V','V','V','V','V','V','V','','',''},'Min',{0,0,0,0,0,0,0,0,0,0,0,0,0,0,0,0,0,0,0,0,0,0,0,0,0,0,0,0,0,0,0,0,0,0,0,0,0,0},'Max',{0,15,1,1,1,5.119375,5.119375,5.119375,5.119375,5.119375,5.119375,5.119375,5.119375,5.119375,5.119375,5.119375,5.119375,5.119375,5.119375,5.119375,5.119375,5.119375,5.119375,0,0,0,5.119375,5.119375,5.119375,5.119375,5.119375,5.119375,5.119375,5.119375,5.119375,0,0,0},'SLDataType',{'SS_DOUBLE','SS_DOUBLE','SS_DOUBLE','SS_DOUBLE','SS_DOUBLE','SS_DOUBLE','SS_DOUBLE','SS_DOUBLE','SS_DOUBLE','SS_DOUBLE','SS_DOUBLE','SS_DOUBLE','SS_DOUBLE','SS_DOUBLE','SS_DOUBLE','SS_DOUBLE','SS_DOUBLE','SS_DOUBLE','SS_DOUBLE','SS_DOUBLE','SS_DOUBLE','SS_DOUBLE','SS_DOUBLE','SS_DOUBLE','SS_DOUBLE','SS_DOUBLE','SS_DOUBLE','SS_DOUBLE','SS_DOUBLE','SS_DOUBLE','SS_DOUBLE','SS_DOUBLE','SS_DOUBLE','SS_DOUBLE','SS_DOUBLE','SS_DOUBLE','SS_DOUBLE','SS_DOUBLE'}),'MsgIdNumFormat',0,'MsgComment',{{''}}),'Version',1.2,'general',struct('isFromLib',0)),'OFF',[]}},'GroupId',{{struct('Group',{{'RTICAN'}},'No',7,'Behavior',{{'NAMECHANGE'}},'BlockType',{{'SINK'}},'NameChangeFlag',0),'OFF',[]}},'SFcnRTICANMessage',{{struct('MsgType','RX','SFcnPortType','Scalar','MsgName','High_V_Batt_Cell_V_Mtrx_3_HV','MsgIdFormat','STD','MsgId',516,'MsgLength',8,'NumSignals',38,'SampleTime',-1,'Signal',struct('SgnName',{'HVBCVM3_CellVltOCVStat','HVBCVM3_CellIndx','HVBCVM3_CellTstSubIDCAct','HVBCVM3_CellTstSubIDBAct','HVBCVM3_CellTstSubIDAAct','HVBCVM3_CellSubIDCVlt','HVBatCell_051','HVBatCell_054','HVBatCell_057','HVBatCell_060','HVBatCell_063','HVBatCell_066','HVBatCell_069','HVBatCell_072','HVBCVM3_CellSubIDBVlt','HVBatCell_050','HVBatCell_053','HVBatCell_056','HVBatCell_059','HVBatCell_062','HVBatCell_065','HVBatCell_068','HVBatCell_071','HVBCVM3_CellSubIDCVltM','HVBCVM3_CellSubIDBVltM','HVBCVM3_CellSubIDAVltM','HVBCVM3_CellSubIDAVlt','HVBatCell_049','HVBatCell_052','HVBatCell_055','HVBatCell_058','HVBatCell_061','HVBatCell_064','HVBatCell_067','HVBatCell_070','HVBCVM3_CellSubIDCVltV','HVBCVM3_CellSubIDBVltV','HVBCVM3_CellSubIDAVltV'},'SgnStartBit',{11,12,16,17,18,19,19,19,19,19,19,19,19,19,32,32,32,32,32,32,32,32,32,45,46,47,48,48,48,48,48,48,48,48,48,61,62,63},'SgnLength',{1,4,1,1,1,13,13,13,13,13,13,13,13,13,13,13,13,13,13,13,13,13,13,1,1,1,13,13,13,13,13,13,13,13,13,1,1,1},'SgnType',{'standard','mode','standard','standard','standard','mode-dependent','mode-dependent','mode-dependent','mode-dependent','mode-dependent','mode-dependent','mode-dependent','mode-dependent','mode-dependent','mode-dependent','mode-dependent','mode-dependent','mode-dependent','mode-dependent','mode-dependent','mode-dependent','mode-dependent','mode-dependent','standard','standard','standard','mode-dependent','mode-dependent','mode-dependent','mode-dependent','mode-dependent','mode-dependent','mode-dependent','mode-dependent','mode-dependent','standard','standard','standard'},'ModeValue',{-1,-1,-1,-1,-1,0,1,3,5,7,9,11,13,15,0,1,3,5,7,9,11,13,15,-1,-1,-1,0,1,3,5,7,9,11,13,15,-1,-1,-1},'DataType',{['unsigned int'],['unsigned int'],['unsigned int'],['unsigned int'],['unsigned int'],['unsigned int'],['unsigned int'],['unsigned int'],['unsigned int'],['unsigned int'],['unsigned int'],['unsigned int'],['unsigned int'],['unsigned int'],['unsigned int'],['unsigned int'],['unsigned int'],['unsigned int'],['unsigned int'],['unsigned int'],['unsigned int'],['unsigned int'],['unsigned int'],['unsigned int'],['unsigned int'],['unsigned int'],['unsigned int'],['unsigned int'],['unsigned int'],['unsigned int'],['unsigned int'],['unsigned int'],['unsigned int'],['unsigned int'],['unsigned int'],['unsigned int'],['unsigned int'],['unsigned int']},'ByteLayout',{['motorola back.'],['motorola back.'],['motorola back.'],['motorola back.'],['motorola back.'],['motorola back.'],['motorola back.'],['motorola back.'],['motorola back.'],['motorola back.'],['motorola back.'],['motorola back.'],['motorola back.'],['motorola back.'],['motorola back.'],['motorola back.'],['motorola back.'],['motorola back.'],['motorola back.'],['motorola back.'],['motorola back.'],['motorola back.'],['motorola back.'],['motorola back.'],['motorola back.'],['motorola back.'],['motorola back.'],['motorola back.'],['motorola back.'],['motorola back.'],['motorola back.'],['motorola back.'],['motorola back.'],['motorola back.'],['motorola back.'],['motorola back.'],['motorola back.'],['motorola back.']},'Factor',{1,1,1,1,1,0.000625,0.000625,0.000625,0.000625,0.000625,0.000625,0.000625,0.000625,0.000625,0.000625,0.000625,0.000625,0.000625,0.000625,0.000625,0.000625,0.000625,0.000625,1,1,1,0.000625,0.000625,0.000625,0.000625,0.000625,0.000625,0.000625,0.000625,0.000625,1,1,1},'Offset',{0,0,0,0,0,0,0,0,0,0,0,0,0,0,0,0,0,0,0,0,0,0,0,0,0,0,0,0,0,0,0,0,0,0,0,0,0,0},'SLDataType',{'SS_DOUBLE','SS_DOUBLE','SS_DOUBLE','SS_DOUBLE','SS_DOUBLE','SS_DOUBLE','SS_DOUBLE','SS_DOUBLE','SS_DOUBLE','SS_DOUBLE','SS_DOUBLE','SS_DOUBLE','SS_DOUBLE','SS_DOUBLE','SS_DOUBLE','SS_DOUBLE','SS_DOUBLE','SS_DOUBLE','SS_DOUBLE','SS_DOUBLE','SS_DOUBLE','SS_DOUBLE','SS_DOUBLE','SS_DOUBLE','SS_DOUBLE','SS_DOUBLE','SS_DOUBLE','SS_DOUBLE','SS_DOUBLE','SS_DOUBLE','SS_DOUBLE','SS_DOUBLE','SS_DOUBLE','SS_DOUBLE','SS_DOUBLE','SS_DOUBLE','SS_DOUBLE','SS_DOUBLE'}),'StatusSelected','no','TimeSelected','no','DeltaTimeSelected','no','BytePortSelected','no','MessageLengthSelected','no','TriggerPort',struct('Selected','no','TriggerType',0),'UserCoding',struct('Selected','no','InterfaceFile','UserDecodingFile','FcnName','UserDecodeFcn','InportSelected','no','InportWidth',1,'OutportSelected','no','OutportWidth',1),'EnablePortSelected','no','UseRXService','no','BoardType','DS4302','BoardNo',1,'ControllerNo',4),'OFF',[]}},'TLCFileName',{{'rtican_rx_message','OFF',[]}})  RTISFcnParameters=struct('SFcnRTICANMessage','struct','TLCFileName','char')  RTIBlockParaDefault=struct('BoardTypeNo',4302,'BoardNo',1,'ChannelNo',1,'Parameters',struct('DataFileSupport',struct('DataFileSelectedMaster',0,'DataFileSelectedLocal',0,'DataFileName','','DataFileDate','','SelectedFile',['<no file selected>']),'Options',struct('StatusSelected',1,'TimeSelected',1,'DeltaTimeSelected',1,'BytePortSelected',0,'MessageLengthSelected',0,'TriggerPort',struct('Selected',0,'TriggerType','rising'),'UserCoding',struct('Selected',0,'InterfaceFile','UserDecodingFile','FcnName','UserDecodeFcn','InportSelected',0,'InportWidth',1,'OutportSelected',0,'OutportWidth',1),'EnablePortSelected',0,'SignalOnPortnameSelected',1,'UseRXService',0),'Message',struct('MsgOnBlocknameSelected',0,'MsgName',['RX Message'],'MsgIdFormat',0,'MsgId',100,'MsgLength',8,'NumSignals',1,'SampleTime',-1,'Signal',struct('SgnName',['RX signal'],'SgnStartBit',0,'SgnLength',8,'SgnType',0,'ModeValue',-1,'DataType',0,'SLDataType','SS_DOUBLE','ByteLayout',0,'Factor',1,'Offset',0,'Min',0,'Max',255,'SgnComment',{{}},'SgnUnit',''),'MsgIdNumFormat',0,'MsgComment',{{''}}),'Version',1.2,'general',struct('isFromLib',1)),'GroupId',struct('Group',{{'RTICAN'}},'No',1,'Behavior',{{'NAMECHANGE'}},'BlockType',{{'SINK'}},'NameChangeFlag',0),'SFcnRTICANMessage',struct('MsgType','RX','MsgName',['RX Message'],'MsgIdFormat','STD','MsgId',100,'MsgLength',8,'NumSignals',1,'SampleTime',-1,'Signal',struct('SgnName',['RX signal'],'SgnStartBit',0,'SgnLength',8,'SgnType','standard','ModeValue',-1,'DataType',['unsigned int'],'ByteLayout',['little endian'],'SLDataType','SS_DOUBLE','Factor',1,'Offset',0),'StatusSelected','yes','TimeSelected','yes','DeltaTimeSelected','yes','BytePortSelected','no','MessageLengthSelected','no','EnablePortSelected','no','UserCoding',struct('Selected','no','InterfaceFile','UserDecodingFile','FcnName','UserDecodeFcn','InportSelected','no','InportWidth',1,'OutportSelected','no','OutportWidth',1),'TriggerPort',struct('Selected','no','TriggerType','rising'),'UseRXService','no','BoardType','DS4302','BoardNo',1,'ControllerNo',1,'SFcnPortType','Scalar'),'TLCFileName','rtican_rx_message')
      settings: AttributesFormatString=Group Id: RTICAN7\n
  High_V_Batt_Cell_V_Mtrx_4_HV1 : rtican/RTICAN Receive (RX)   SystemSampleTime=-1  Reserved1=[]  Reserved2=[]  Reserved3=[]  Reserved4=[]  SfcnMessage=[]  Msg_Struct=[]  BoardTypeNo=[]  BoardNo=[]  ChannelNo=[]  Parameters=[]  DialogFcn=[]  UnitName=[]  Revision=[]  UnitValues=[]  DSProperties=struct('RTI',struct('Version',uint32(5),'BlockType',struct('isSLSource',uint8(1),'isSLSink',uint8(1),'isHWSource',uint8(0),'isHWSink',uint8(0),'isSetup',uint8(0),'isInline',uint8(1),'isNonInline',uint8(0),'isInterrupt',uint8(0),'isChannelwise',uint8(0)),'IOBoardType','RTICAN','UnitType','MESSAGE','Identifier','RX','DialogType','MSVC','BlockSet','RTICAN','SlaveProcessor','CAN'))  RTIBlockInterface=struct('OutputPortsWidth',int32([1 1 1 1 1 1 1 1 1 1 1 1 1 1 1 1 1 1 1 1 1 1 1 1 1 1 1 1 1 1 1 1 1 1 1 1 1 1]),'OutputPortsActive',[1 1 1 1 1 1 1 1 1 1 1 1 1 1 1 1 1 1 1 1 1 1 1 1 1 1 1 1 1 1 1 1 1 1 1 1 1 1],'OutputPortsName',{{'HVBCVM4_CellVltOCVStat','HVBCVM4_CellIndx','HVBCVM4_CellTstSubIDCAct','HVBCVM4_CellTstSubIDBAct','HVBCVM4_CellTstSubIDAAct','HVBCVM4_CellSubIDCVlt','HVBatCell_075','HVBatCell_078','HVBatCell_081','HVBatCell_084','HVBatCell_087','HVBatCell_090','HVBatCell_093','HVBatCell_096','HVBCVM4_CellSubIDBVlt','HVBatCell_074','HVBatCell_077','HVBatCell_080','HVBatCell_083','HVBatCell_086','HVBatCell_089','HVBatCell_092','HVBatCell_095','HVBCVM4_CellSubIDCVltM','HVBCVM4_CellSubIDBVltM','HVBCVM4_CellSubIDAVltM','HVBCVM4_CellSubIDAVlt','HVBatCell_073','HVBatCell_076','HVBatCell_079','HVBatCell_082','HVBatCell_085','HVBatCell_088','HVBatCell_091','HVBatCell_094','HVBCVM4_CellSubIDCVltV','HVBCVM4_CellSubIDBVltV','HVBCVM4_CellSubIDAVltV'}},'OutputPortsDataType',{{'SS_DOUBLE','SS_DOUBLE','SS_DOUBLE','SS_DOUBLE','SS_DOUBLE','SS_DOUBLE','SS_DOUBLE','SS_DOUBLE','SS_DOUBLE','SS_DOUBLE','SS_DOUBLE','SS_DOUBLE','SS_DOUBLE','SS_DOUBLE','SS_DOUBLE','SS_DOUBLE','SS_DOUBLE','SS_DOUBLE','SS_DOUBLE','SS_DOUBLE','SS_DOUBLE','SS_DOUBLE','SS_DOUBLE','SS_DOUBLE','SS_DOUBLE','SS_DOUBLE','SS_DOUBLE','SS_DOUBLE','SS_DOUBLE','SS_DOUBLE','SS_DOUBLE','SS_DOUBLE','SS_DOUBLE','SS_DOUBLE','SS_DOUBLE','SS_DOUBLE','SS_DOUBLE','SS_DOUBLE'}},'OutputPortsLabel',{{'HVBCVM4_CellVltOCVStat','HVBCVM4_CellIndx','HVBCVM4_CellTstSubIDCAct','HVBCVM4_CellTstSubIDBAct','HVBCVM4_CellTstSubIDAAct','HVBCVM4_CellSubIDCVlt','HVBatCell_075','HVBatCell_078','HVBatCell_081','HVBatCell_084','HVBatCell_087','HVBatCell_090','HVBatCell_093','HVBatCell_096','HVBCVM4_CellSubIDBVlt','HVBatCell_074','HVBatCell_077','HVBatCell_080','HVBatCell_083','HVBatCell_086','HVBatCell_089','HVBatCell_092','HVBatCell_095','HVBCVM4_CellSubIDCVltM','HVBCVM4_CellSubIDBVltM','HVBCVM4_CellSubIDAVltM','HVBCVM4_CellSubIDAVlt','HVBatCell_073','HVBatCell_076','HVBatCell_079','HVBatCell_082','HVBatCell_085','HVBatCell_088','HVBatCell_091','HVBatCell_094','HVBCVM4_CellSubIDCVltV','HVBCVM4_CellSubIDBVltV','HVBCVM4_CellSubIDAVltV'}},'OutputPortsLabelMode','ON','InputPortsWidth',int32(0),'InputPortsActive',0,'DialogFcn','rtican_message_interface_gui','BlockDisplay',{{'','center'}},'IconTransparency','on','ParameterTunableNames',{{}},'InitLevel',3,'BlockName',struct('Token',{{'High_V_Batt_Cell_V_Mtrx_4_HV'}}),'SampleTime',{{-1}},'TriggerPort',{{'none'}},'EnablePort',{{'none'}})  RTIBlockParameters=struct('BoardTypeNo',{{4302,'OFF',[]}},'BoardNo',{{1,'ON',[1 16]}},'ChannelNo',{{4,'ON',[1 4]}},'Parameters',{{struct('DataFileSupport',struct('DataFileSelectedMaster',1,'DataFileSelectedLocal',1,'DataFileName',['c:\data\databases\6.4.1\globala - hv.dbc|c:\data\testing\dbc\globala - hvdmx112.dbc|'],'DataFileDate',{{{['06-Jan-2012 10:17:38']},{['10-May-2011 15:46:00']}}},'SelectedFile',['dbc\globala - hvdmx112.dbc']),'Options',struct('StatusSelected',0,'TimeSelected',0,'DeltaTimeSelected',0,'BytePortSelected',0,'MessageLengthSelected',0,'TriggerPort',struct('Selected',0,'TriggerType',0),'UserCoding',struct('Selected',0,'InterfaceFile','UserDecodingFile','FcnName','UserDecodeFcn','InportSelected',0,'InportWidth',1,'OutportSelected',0,'OutportWidth',1),'EnablePortSelected',0,'SignalOnPortnameSelected',1,'UseRXService',0),'Message',struct('MsgOnBlocknameSelected',1,'MsgName','High_V_Batt_Cell_V_Mtrx_4_HV','MsgIdFormat',0,'MsgId',518,'MsgLength',8,'NumSignals',38,'SampleTime',-1,'Signal',struct('SgnName',{'HVBCVM4_CellVltOCVStat','HVBCVM4_CellIndx','HVBCVM4_CellTstSubIDCAct','HVBCVM4_CellTstSubIDBAct','HVBCVM4_CellTstSubIDAAct','HVBCVM4_CellSubIDCVlt','HVBatCell_075','HVBatCell_078','HVBatCell_081','HVBatCell_084','HVBatCell_087','HVBatCell_090','HVBatCell_093','HVBatCell_096','HVBCVM4_CellSubIDBVlt','HVBatCell_074','HVBatCell_077','HVBatCell_080','HVBatCell_083','HVBatCell_086','HVBatCell_089','HVBatCell_092','HVBatCell_095','HVBCVM4_CellSubIDCVltM','HVBCVM4_CellSubIDBVltM','HVBCVM4_CellSubIDAVltM','HVBCVM4_CellSubIDAVlt','HVBatCell_073','HVBatCell_076','HVBatCell_079','HVBatCell_082','HVBatCell_085','HVBatCell_088','HVBatCell_091','HVBatCell_094','HVBCVM4_CellSubIDCVltV','HVBCVM4_CellSubIDBVltV','HVBCVM4_CellSubIDAVltV'},'SgnStartBit',{11,12,16,17,18,19,19,19,19,19,19,19,19,19,32,32,32,32,32,32,32,32,32,45,46,47,48,48,48,48,48,48,48,48,48,61,62,63},'SgnLength',{1,4,1,1,1,13,13,13,13,13,13,13,13,13,13,13,13,13,13,13,13,13,13,1,1,1,13,13,13,13,13,13,13,13,13,1,1,1},'SgnType',{0,1,0,0,0,2,2,2,2,2,2,2,2,2,2,2,2,2,2,2,2,2,2,0,0,0,2,2,2,2,2,2,2,2,2,0,0,0},'ModeValue',{-1,-1,-1,-1,-1,0,1,3,5,7,9,11,13,15,0,1,3,5,7,9,11,13,15,-1,-1,-1,0,1,3,5,7,9,11,13,15,-1,-1,-1},'DataType',{0,0,0,0,0,0,0,0,0,0,0,0,0,0,0,0,0,0,0,0,0,0,0,0,0,0,0,0,0,0,0,0,0,0,0,0,0,0},'ByteLayout',{2,2,2,2,2,2,2,2,2,2,2,2,2,2,2,2,2,2,2,2,2,2,2,2,2,2,2,2,2,2,2,2,2,2,2,2,2,2},'Factor',{1,1,1,1,1,0.000625,0.000625,0.000625,0.000625,0.000625,0.000625,0.000625,0.000625,0.000625,0.000625,0.000625,0.000625,0.000625,0.000625,0.000625,0.000625,0.000625,0.000625,1,1,1,0.000625,0.000625,0.000625,0.000625,0.000625,0.000625,0.000625,0.000625,0.000625,1,1,1},'Offset',{0,0,0,0,0,0,0,0,0,0,0,0,0,0,0,0,0,0,0,0,0,0,0,0,0,0,0,0,0,0,0,0,0,0,0,0,0,0},'SgnComment',{{''},{''},{''},{''},{''},{''},{''},{''},{''},{''},{''},{''},{''},{''},{''},{''},{''},{''},{''},{''},{''},{''},{''},{''},{''},{''},{''},{''},{''},{''},{''},{''},{''},{''},{''},{''},{''},{''}},'SgnUnit',{'','','','','','V','V','V','V','V','V','V','V','V','V','V','V','V','V','V','V','V','V','','','','V','V','V','V','V','V','V','V','V','','',''},'Min',{0,0,0,0,0,0,0,0,0,0,0,0,0,0,0,0,0,0,0,0,0,0,0,0,0,0,0,0,0,0,0,0,0,0,0,0,0,0},'Max',{0,15,1,1,1,5.119375,5.119375,5.119375,5.119375,5.119375,5.119375,5.119375,5.119375,5.119375,5.119375,5.119375,5.119375,5.119375,5.119375,5.119375,5.119375,5.119375,5.119375,0,0,0,5.119375,5.119375,5.119375,5.119375,5.119375,5.119375,5.119375,5.119375,5.119375,0,0,0},'SLDataType',{'SS_DOUBLE','SS_DOUBLE','SS_DOUBLE','SS_DOUBLE','SS_DOUBLE','SS_DOUBLE','SS_DOUBLE','SS_DOUBLE','SS_DOUBLE','SS_DOUBLE','SS_DOUBLE','SS_DOUBLE','SS_DOUBLE','SS_DOUBLE','SS_DOUBLE','SS_DOUBLE','SS_DOUBLE','SS_DOUBLE','SS_DOUBLE','SS_DOUBLE','SS_DOUBLE','SS_DOUBLE','SS_DOUBLE','SS_DOUBLE','SS_DOUBLE','SS_DOUBLE','SS_DOUBLE','SS_DOUBLE','SS_DOUBLE','SS_DOUBLE','SS_DOUBLE','SS_DOUBLE','SS_DOUBLE','SS_DOUBLE','SS_DOUBLE','SS_DOUBLE','SS_DOUBLE','SS_DOUBLE'}),'MsgIdNumFormat',0,'MsgComment',{{''}}),'Version',1.2,'general',struct('isFromLib',0)),'OFF',[]}},'GroupId',{{struct('Group',{{'RTICAN'}},'No',7,'Behavior',{{'NAMECHANGE'}},'BlockType',{{'SINK'}},'NameChangeFlag',0),'OFF',[]}},'SFcnRTICANMessage',{{struct('MsgType','RX','SFcnPortType','Scalar','MsgName','High_V_Batt_Cell_V_Mtrx_4_HV','MsgIdFormat','STD','MsgId',518,'MsgLength',8,'NumSignals',38,'SampleTime',-1,'Signal',struct('SgnName',{'HVBCVM4_CellVltOCVStat','HVBCVM4_CellIndx','HVBCVM4_CellTstSubIDCAct','HVBCVM4_CellTstSubIDBAct','HVBCVM4_CellTstSubIDAAct','HVBCVM4_CellSubIDCVlt','HVBatCell_075','HVBatCell_078','HVBatCell_081','HVBatCell_084','HVBatCell_087','HVBatCell_090','HVBatCell_093','HVBatCell_096','HVBCVM4_CellSubIDBVlt','HVBatCell_074','HVBatCell_077','HVBatCell_080','HVBatCell_083','HVBatCell_086','HVBatCell_089','HVBatCell_092','HVBatCell_095','HVBCVM4_CellSubIDCVltM','HVBCVM4_CellSubIDBVltM','HVBCVM4_CellSubIDAVltM','HVBCVM4_CellSubIDAVlt','HVBatCell_073','HVBatCell_076','HVBatCell_079','HVBatCell_082','HVBatCell_085','HVBatCell_088','HVBatCell_091','HVBatCell_094','HVBCVM4_CellSubIDCVltV','HVBCVM4_CellSubIDBVltV','HVBCVM4_CellSubIDAVltV'},'SgnStartBit',{11,12,16,17,18,19,19,19,19,19,19,19,19,19,32,32,32,32,32,32,32,32,32,45,46,47,48,48,48,48,48,48,48,48,48,61,62,63},'SgnLength',{1,4,1,1,1,13,13,13,13,13,13,13,13,13,13,13,13,13,13,13,13,13,13,1,1,1,13,13,13,13,13,13,13,13,13,1,1,1},'SgnType',{'standard','mode','standard','standard','standard','mode-dependent','mode-dependent','mode-dependent','mode-dependent','mode-dependent','mode-dependent','mode-dependent','mode-dependent','mode-dependent','mode-dependent','mode-dependent','mode-dependent','mode-dependent','mode-dependent','mode-dependent','mode-dependent','mode-dependent','mode-dependent','standard','standard','standard','mode-dependent','mode-dependent','mode-dependent','mode-dependent','mode-dependent','mode-dependent','mode-dependent','mode-dependent','mode-dependent','standard','standard','standard'},'ModeValue',{-1,-1,-1,-1,-1,0,1,3,5,7,9,11,13,15,0,1,3,5,7,9,11,13,15,-1,-1,-1,0,1,3,5,7,9,11,13,15,-1,-1,-1},'DataType',{['unsigned int'],['unsigned int'],['unsigned int'],['unsigned int'],['unsigned int'],['unsigned int'],['unsigned int'],['unsigned int'],['unsigned int'],['unsigned int'],['unsigned int'],['unsigned int'],['unsigned int'],['unsigned int'],['unsigned int'],['unsigned int'],['unsigned int'],['unsigned int'],['unsigned int'],['unsigned int'],['unsigned int'],['unsigned int'],['unsigned int'],['unsigned int'],['unsigned int'],['unsigned int'],['unsigned int'],['unsigned int'],['unsigned int'],['unsigned int'],['unsigned int'],['unsigned int'],['unsigned int'],['unsigned int'],['unsigned int'],['unsigned int'],['unsigned int'],['unsigned int']},'ByteLayout',{['motorola back.'],['motorola back.'],['motorola back.'],['motorola back.'],['motorola back.'],['motorola back.'],['motorola back.'],['motorola back.'],['motorola back.'],['motorola back.'],['motorola back.'],['motorola back.'],['motorola back.'],['motorola back.'],['motorola back.'],['motorola back.'],['motorola back.'],['motorola back.'],['motorola back.'],['motorola back.'],['motorola back.'],['motorola back.'],['motorola back.'],['motorola back.'],['motorola back.'],['motorola back.'],['motorola back.'],['motorola back.'],['motorola back.'],['motorola back.'],['motorola back.'],['motorola back.'],['motorola back.'],['motorola back.'],['motorola back.'],['motorola back.'],['motorola back.'],['motorola back.']},'Factor',{1,1,1,1,1,0.000625,0.000625,0.000625,0.000625,0.000625,0.000625,0.000625,0.000625,0.000625,0.000625,0.000625,0.000625,0.000625,0.000625,0.000625,0.000625,0.000625,0.000625,1,1,1,0.000625,0.000625,0.000625,0.000625,0.000625,0.000625,0.000625,0.000625,0.000625,1,1,1},'Offset',{0,0,0,0,0,0,0,0,0,0,0,0,0,0,0,0,0,0,0,0,0,0,0,0,0,0,0,0,0,0,0,0,0,0,0,0,0,0},'SLDataType',{'SS_DOUBLE','SS_DOUBLE','SS_DOUBLE','SS_DOUBLE','SS_DOUBLE','SS_DOUBLE','SS_DOUBLE','SS_DOUBLE','SS_DOUBLE','SS_DOUBLE','SS_DOUBLE','SS_DOUBLE','SS_DOUBLE','SS_DOUBLE','SS_DOUBLE','SS_DOUBLE','SS_DOUBLE','SS_DOUBLE','SS_DOUBLE','SS_DOUBLE','SS_DOUBLE','SS_DOUBLE','SS_DOUBLE','SS_DOUBLE','SS_DOUBLE','SS_DOUBLE','SS_DOUBLE','SS_DOUBLE','SS_DOUBLE','SS_DOUBLE','SS_DOUBLE','SS_DOUBLE','SS_DOUBLE','SS_DOUBLE','SS_DOUBLE','SS_DOUBLE','SS_DOUBLE','SS_DOUBLE'}),'StatusSelected','no','TimeSelected','no','DeltaTimeSelected','no','BytePortSelected','no','MessageLengthSelected','no','TriggerPort',struct('Selected','no','TriggerType',0),'UserCoding',struct('Selected','no','InterfaceFile','UserDecodingFile','FcnName','UserDecodeFcn','InportSelected','no','InportWidth',1,'OutportSelected','no','OutportWidth',1),'EnablePortSelected','no','UseRXService','no','BoardType','DS4302','BoardNo',1,'ControllerNo',4),'OFF',[]}},'TLCFileName',{{'rtican_rx_message','OFF',[]}})  RTISFcnParameters=struct('SFcnRTICANMessage','struct','TLCFileName','char')  RTIBlockParaDefault=struct('BoardTypeNo',4302,'BoardNo',1,'ChannelNo',1,'Parameters',struct('DataFileSupport',struct('DataFileSelectedMaster',0,'DataFileSelectedLocal',0,'DataFileName','','DataFileDate','','SelectedFile',['<no file selected>']),'Options',struct('StatusSelected',1,'TimeSelected',1,'DeltaTimeSelected',1,'BytePortSelected',0,'MessageLengthSelected',0,'TriggerPort',struct('Selected',0,'TriggerType','rising'),'UserCoding',struct('Selected',0,'InterfaceFile','UserDecodingFile','FcnName','UserDecodeFcn','InportSelected',0,'InportWidth',1,'OutportSelected',0,'OutportWidth',1),'EnablePortSelected',0,'SignalOnPortnameSelected',1,'UseRXService',0),'Message',struct('MsgOnBlocknameSelected',0,'MsgName',['RX Message'],'MsgIdFormat',0,'MsgId',100,'MsgLength',8,'NumSignals',1,'SampleTime',-1,'Signal',struct('SgnName',['RX signal'],'SgnStartBit',0,'SgnLength',8,'SgnType',0,'ModeValue',-1,'DataType',0,'SLDataType','SS_DOUBLE','ByteLayout',0,'Factor',1,'Offset',0,'Min',0,'Max',255,'SgnComment',{{}},'SgnUnit',''),'MsgIdNumFormat',0,'MsgComment',{{''}}),'Version',1.2,'general',struct('isFromLib',1)),'GroupId',struct('Group',{{'RTICAN'}},'No',1,'Behavior',{{'NAMECHANGE'}},'BlockType',{{'SINK'}},'NameChangeFlag',0),'SFcnRTICANMessage',struct('MsgType','RX','MsgName',['RX Message'],'MsgIdFormat','STD','MsgId',100,'MsgLength',8,'NumSignals',1,'SampleTime',-1,'Signal',struct('SgnName',['RX signal'],'SgnStartBit',0,'SgnLength',8,'SgnType','standard','ModeValue',-1,'DataType',['unsigned int'],'ByteLayout',['little endian'],'SLDataType','SS_DOUBLE','Factor',1,'Offset',0),'StatusSelected','yes','TimeSelected','yes','DeltaTimeSelected','yes','BytePortSelected','no','MessageLengthSelected','no','EnablePortSelected','no','UserCoding',struct('Selected','no','InterfaceFile','UserDecodingFile','FcnName','UserDecodeFcn','InportSelected','no','InportWidth',1,'OutportSelected','no','OutportWidth',1),'TriggerPort',struct('Selected','no','TriggerType','rising'),'UseRXService','no','BoardType','DS4302','BoardNo',1,'ControllerNo',1,'SFcnPortType','Scalar'),'TLCFileName','rtican_rx_message')
      settings: AttributesFormatString=Group Id: RTICAN7\n
  MinMax{1,3,5,7,11} (5 alike) : MinMax  Function=max  OutDataType=fixdt(1, 16)  OutScaling=2^0
  MinMax{2,4,6,9..10} (5 alike) : MinMax  OutDataType=sfix(16)  OutScaling=2^0
  Subsystem : Subsystem
  Sum of Elements{,1..3} (4 alike) : Sum  Inputs=+  OutDataType=fixdt(1, 16)  OutScaling=2^-10
  SumofCells : Sum  Inputs=++++  OutDataType=fixdt(1, 16)  OutScaling=2^-10
  Terminator_{1..14,18..31,35..62} (56 alike) : Terminator
  SumCells : Outport  OutDataType=fixdt(1, 16)  OutScaling=2^0
  MinCell : Outport  Port=2  OutDataType=fixdt(1, 16)  OutScaling=2^0
  MaxCell : Outport  Port=3  OutDataType=fixdt(1, 16)  OutScaling=2^0
  MinSection_PackEquivalent : Outport  Port=4  OutDataType=fixdt(1, 16)  OutScaling=2^0
  wires:
  [Msg200] -> SumofCells/1
  [Msg202] -> SumofCells/2
  [Msg204] -> SumofCells/3
  [Msg206] -> SumofCells/4
  SumofCells/1 -> Gain5/1
  Bus Creator/1 -> MinMax1/1, MinMax10/1, Sum of Elements/1, [CellMatrixOne]
  Sum of Elements/1 -> [Msg200]
  MinMax1/1 -> [MaxMsg200]
  Bus Creator1/1 -> Sum of Elements1/1, MinMax2/1, MinMax3/1, [CellMatrixTwo]
  High_V_Batt_Cell_V_Mtrx_2_HV1/7 -> Bus Creator1/1  "HVBatCell_027"
  High_V_Batt_Cell_V_Mtrx_2_HV1/8 -> Bus Creator1/2  "HVBatCell_030"
  High_V_Batt_Cell_V_Mtrx_2_HV1/9 -> Bus Creator1/3  "HVBatCell_033"
  High_V_Batt_Cell_V_Mtrx_2_HV1/10 -> Bus Creator1/4  "HVBatCell_036"
  High_V_Batt_Cell_V_Mtrx_2_HV1/11 -> Bus Creator1/5  "HVBatCell_039"
  High_V_Batt_Cell_V_Mtrx_2_HV1/12 -> Bus Creator1/6  "HVBatCell_042"
  High_V_Batt_Cell_V_Mtrx_2_HV1/13 -> Bus Creator1/7  "HVBatCell_045"
  High_V_Batt_Cell_V_Mtrx_2_HV1/14 -> Bus Creator1/8  "HVBatCell_048"
  High_V_Batt_Cell_V_Mtrx_2_HV1/16 -> Bus Creator1/9  "HVBatCell_026"
  High_V_Batt_Cell_V_Mtrx_2_HV1/17 -> Bus Creator1/10  "HVBatCell_029"
  High_V_Batt_Cell_V_Mtrx_2_HV1/18 -> Bus Creator1/11  "HVBatCell_032"
  High_V_Batt_Cell_V_Mtrx_2_HV1/19 -> Bus Creator1/12  "HVBatCell_035"
  High_V_Batt_Cell_V_Mtrx_2_HV1/20 -> Bus Creator1/13  "HVBatCell_038"
  High_V_Batt_Cell_V_Mtrx_2_HV1/21 -> Bus Creator1/14  "HVBatCell_041"
  High_V_Batt_Cell_V_Mtrx_2_HV1/22 -> Bus Creator1/15  "HVBatCell_044"
  High_V_Batt_Cell_V_Mtrx_2_HV1/23 -> Bus Creator1/16  "HVBatCell_047"
  High_V_Batt_Cell_V_Mtrx_2_HV1/28 -> Bus Creator1/17  "HVBatCell_025"
  High_V_Batt_Cell_V_Mtrx_2_HV1/29 -> Bus Creator1/18  "HVBatCell_028"
  High_V_Batt_Cell_V_Mtrx_2_HV1/30 -> Bus Creator1/19  "HVBatCell_031"
  High_V_Batt_Cell_V_Mtrx_2_HV1/31 -> Bus Creator1/20  "HVBatCell_034"
  High_V_Batt_Cell_V_Mtrx_2_HV1/32 -> Bus Creator1/21  "HVBatCell_037"
  High_V_Batt_Cell_V_Mtrx_2_HV1/33 -> Bus Creator1/22  "HVBatCell_040"
  High_V_Batt_Cell_V_Mtrx_2_HV1/34 -> Bus Creator1/23  "HVBatCell_043"
  High_V_Batt_Cell_V_Mtrx_2_HV1/35 -> Bus Creator1/24  "HVBatCell_046"
  Sum of Elements1/1 -> [Msg202]
  MinMax2/1 -> Gain1/1
  MinMax3/1 -> [MaxMsg202]
  High_V_Batt_Cell_V_Mtrx_3_HV1/7 -> Bus Creator2/1  "HVBatCell_051"
  High_V_Batt_Cell_V_Mtrx_3_HV1/8 -> Bus Creator2/2  "HVBatCell_054"
  High_V_Batt_Cell_V_Mtrx_3_HV1/9 -> Bus Creator2/3  "HVBatCell_057"
  High_V_Batt_Cell_V_Mtrx_3_HV1/10 -> Bus Creator2/4  "HVBatCell_060"
  High_V_Batt_Cell_V_Mtrx_3_HV1/11 -> Bus Creator2/5  "HVBatCell_063"
  High_V_Batt_Cell_V_Mtrx_3_HV1/12 -> Bus Creator2/6  "HVBatCell_066"
  High_V_Batt_Cell_V_Mtrx_3_HV1/13 -> Bus Creator2/7  "HVBatCell_069"
  High_V_Batt_Cell_V_Mtrx_3_HV1/14 -> Bus Creator2/8  "HVBatCell_072"
  High_V_Batt_Cell_V_Mtrx_3_HV1/16 -> Bus Creator2/9  "HVBatCell_050"
  High_V_Batt_Cell_V_Mtrx_3_HV1/17 -> Bus Creator2/10  "HVBatCell_053"
  High_V_Batt_Cell_V_Mtrx_3_HV1/18 -> Bus Creator2/11  "HVBatCell_056"
  High_V_Batt_Cell_V_Mtrx_3_HV1/19 -> Bus Creator2/12  "HVBatCell_059"
  High_V_Batt_Cell_V_Mtrx_3_HV1/20 -> Bus Creator2/13  "HVBatCell_062"
  High_V_Batt_Cell_V_Mtrx_3_HV1/21 -> Bus Creator2/14  "HVBatCell_065"
  High_V_Batt_Cell_V_Mtrx_3_HV1/22 -> Bus Creator2/15  "HVBatCell_068"
  High_V_Batt_Cell_V_Mtrx_3_HV1/23 -> Bus Creator2/16  "HVBatCell_071"
  High_V_Batt_Cell_V_Mtrx_3_HV1/28 -> Bus Creator2/17  "HVBatCell_049"
  High_V_Batt_Cell_V_Mtrx_3_HV1/29 -> Bus Creator2/18  "HVBatCell_052"
  High_V_Batt_Cell_V_Mtrx_3_HV1/30 -> Bus Creator2/19  "HVBatCell_055"
  High_V_Batt_Cell_V_Mtrx_3_HV1/31 -> Bus Creator2/20  "HVBatCell_058"
  High_V_Batt_Cell_V_Mtrx_3_HV1/32 -> Bus Creator2/21  "HVBatCell_061"
  High_V_Batt_Cell_V_Mtrx_3_HV1/33 -> Bus Creator2/22  "HVBatCell_064"
  High_V_Batt_Cell_V_Mtrx_3_HV1/34 -> Bus Creator2/23  "HVBatCell_067"
  High_V_Batt_Cell_V_Mtrx_3_HV1/35 -> Bus Creator2/24  "HVBatCell_070"
  Bus Creator2/1 -> MinMax4/1, Sum of Elements2/1, [CellMatrixThree], MinMax5/1
  Sum of Elements2/1 -> [Msg204]
  MinMax5/1 -> [MaxMsg204]
  High_V_Batt_Cell_V_Mtrx_4_HV1/7 -> Bus Creator3/1  "HVBatCell_075"
  High_V_Batt_Cell_V_Mtrx_4_HV1/8 -> Bus Creator3/2  "HVBatCell_078"
  High_V_Batt_Cell_V_Mtrx_4_HV1/9 -> Bus Creator3/3  "HVBatCell_081"
  High_V_Batt_Cell_V_Mtrx_4_HV1/10 -> Bus Creator3/4  "HVBatCell_084"
  High_V_Batt_Cell_V_Mtrx_4_HV1/11 -> Bus Creator3/5  "HVBatCell_087"
  High_V_Batt_Cell_V_Mtrx_4_HV1/12 -> Bus Creator3/6  "HVBatCell_090"
  High_V_Batt_Cell_V_Mtrx_4_HV1/13 -> Bus Creator3/7  "HVBatCell_093"
  High_V_Batt_Cell_V_Mtrx_4_HV1/14 -> Bus Creator3/8  "HVBatCell_096"
  High_V_Batt_Cell_V_Mtrx_4_HV1/16 -> Bus Creator3/9  "HVBatCell_074"
  High_V_Batt_Cell_V_Mtrx_4_HV1/17 -> Bus Creator3/10  "HVBatCell_077"
  High_V_Batt_Cell_V_Mtrx_4_HV1/18 -> Bus Creator3/11  "HVBatCell_080"
  High_V_Batt_Cell_V_Mtrx_4_HV1/19 -> Bus Creator3/12  "HVBatCell_083"
  High_V_Batt_Cell_V_Mtrx_4_HV1/20 -> Bus Creator3/13  "HVBatCell_086"
  High_V_Batt_Cell_V_Mtrx_4_HV1/21 -> Bus Creator3/14  "HVBatCell_089"
  High_V_Batt_Cell_V_Mtrx_4_HV1/22 -> Bus Creator3/15  "HVBatCell_092"
  High_V_Batt_Cell_V_Mtrx_4_HV1/23 -> Bus Creator3/16  "HVBatCell_095"
  High_V_Batt_Cell_V_Mtrx_4_HV1/28 -> Bus Creator3/17  "HVBatCell_073"
  High_V_Batt_Cell_V_Mtrx_4_HV1/29 -> Bus Creator3/18  "HVBatCell_076"
  High_V_Batt_Cell_V_Mtrx_4_HV1/30 -> Bus Creator3/19  "HVBatCell_079"
  High_V_Batt_Cell_V_Mtrx_4_HV1/31 -> Bus Creator3/20  "HVBatCell_082"
  High_V_Batt_Cell_V_Mtrx_4_HV1/32 -> Bus Creator3/21  "HVBatCell_085"
  High_V_Batt_Cell_V_Mtrx_4_HV1/33 -> Bus Creator3/22  "HVBatCell_088"
  High_V_Batt_Cell_V_Mtrx_4_HV1/34 -> Bus Creator3/23  "HVBatCell_091"
  High_V_Batt_Cell_V_Mtrx_4_HV1/35 -> Bus Creator3/24  "HVBatCell_094"
  Sum of Elements3/1 -> [Msg206]
  Bus Creator3/1 -> Sum of Elements3/1, MinMax6/1, MinMax7/1, [CellMatrixFour]
  MinMax6/1 -> Gain3/1
  MinMax7/1 -> [MaxMsg206]
  [MinMsg200] -> Bus Creator5/1
  [MinMsg202] -> Bus Creator5/2
  [MinMsg206] -> Bus Creator5/4
  [MinMsg204] -> Bus Creator5/3
  Bus Creator5/1 -> MinMax9/1
  MinMax9/1 -> MinCell/1
  [MaxMsg200] -> Bus Creator6/1
  [MaxMsg202] -> Bus Creator6/2
  [MaxMsg206] -> Bus Creator6/4
  [MaxMsg204] -> Bus Creator6/3
  Bus Creator6/1 -> MinMax11/1
  MinMax11/1 -> MaxCell/1
  High_V_Batt_Cell_V_Mtrx_1_HV1/7 -> Bus Creator/1  "HVBatCell_003"
  High_V_Batt_Cell_V_Mtrx_1_HV1/8 -> Bus Creator/2  "HVBatCell_006"
  High_V_Batt_Cell_V_Mtrx_1_HV1/9 -> Bus Creator/3  "HVBatCell_009"
  High_V_Batt_Cell_V_Mtrx_1_HV1/10 -> Bus Creator/4  "HVBatCell_012"
  High_V_Batt_Cell_V_Mtrx_1_HV1/11 -> Bus Creator/5  "HVBatCell_015"
  High_V_Batt_Cell_V_Mtrx_1_HV1/12 -> Bus Creator/6  "HVBatCell_018"
  High_V_Batt_Cell_V_Mtrx_1_HV1/13 -> Bus Creator/7  "HVBatCell_021"
  High_V_Batt_Cell_V_Mtrx_1_HV1/14 -> Bus Creator/8  "HVBatCell_024"
  High_V_Batt_Cell_V_Mtrx_1_HV1/16 -> Bus Creator/9  "HVBatCell_002"
  High_V_Batt_Cell_V_Mtrx_1_HV1/17 -> Bus Creator/10  "HVBatCell_005"
  High_V_Batt_Cell_V_Mtrx_1_HV1/18 -> Bus Creator/11  "HVBatCell_008"
  High_V_Batt_Cell_V_Mtrx_1_HV1/19 -> Bus Creator/12  "HVBatCell_011"
  High_V_Batt_Cell_V_Mtrx_1_HV1/20 -> Bus Creator/13  "HVBatCell_014"
  High_V_Batt_Cell_V_Mtrx_1_HV1/21 -> Bus Creator/14  "HVBatCell_017"
  High_V_Batt_Cell_V_Mtrx_1_HV1/22 -> Bus Creator/15  "HVBatCell_020"
  High_V_Batt_Cell_V_Mtrx_1_HV1/23 -> Bus Creator/16  "HVBatCell_023"
  High_V_Batt_Cell_V_Mtrx_1_HV1/28 -> Bus Creator/17  "HVBatCell_001"
  High_V_Batt_Cell_V_Mtrx_1_HV1/29 -> Bus Creator/18  "HVBatCell_004"
  High_V_Batt_Cell_V_Mtrx_1_HV1/30 -> Bus Creator/19  "HVBatCell_007"
  High_V_Batt_Cell_V_Mtrx_1_HV1/31 -> Bus Creator/20  "HVBatCell_010"
  High_V_Batt_Cell_V_Mtrx_1_HV1/32 -> Bus Creator/21  "HVBatCell_013"
  High_V_Batt_Cell_V_Mtrx_1_HV1/33 -> Bus Creator/22  "HVBatCell_016"
  High_V_Batt_Cell_V_Mtrx_1_HV1/34 -> Bus Creator/23  "HVBatCell_019"
  High_V_Batt_Cell_V_Mtrx_1_HV1/35 -> Bus Creator/24  "HVBatCell_022"
  Gain/1 -> [MinMsg200], Compare To Zero/1
  MinMax10/1 -> Gain/1
  Gain1/1 -> [MinMsg202], Compare To Zero1/1
  MinMax4/1 -> Gain2/1
  Gain2/1 -> [MinMsg204], Compare To Zero2/1
  Gain3/1 -> [MinMsg206], Compare To Zero3/1
  Compare To Zero/1 -> [ch]
  Compare To Zero1/1 -> [ch1]
  Compare To Zero2/1 -> [ch2]
  Compare To Zero3/1 -> [ch3]
  High_V_Batt_Cell_V_Mtrx_1_HV1/1 -> Terminator_1/1  "HVBCVM1_CellOCVStat"
  High_V_Batt_Cell_V_Mtrx_1_HV1/2 -> Terminator_2/1  "HVBCVM1_CellIndx"
  High_V_Batt_Cell_V_Mtrx_1_HV1/3 -> Terminator_3/1  "HVBCVM1_CellTstSubIDCAct"
  High_V_Batt_Cell_V_Mtrx_1_HV1/4 -> Terminator_4/1  "HVBCVM1_CellTstSubIDBAct"
  High_V_Batt_Cell_V_Mtrx_1_HV1/5 -> Terminator_5/1  "HVBCVM1_CellTstSubIDAAct"
  High_V_Batt_Cell_V_Mtrx_1_HV1/6 -> Terminator_6/1  "HVBCVM1_CellSubIDCVlt"
  High_V_Batt_Cell_V_Mtrx_1_HV1/15 -> Terminator_7/1  "HVBCVM1_CellSubIDBVlt"
  High_V_Batt_Cell_V_Mtrx_1_HV1/24 -> Terminator_8/1  "HVBCVM1_CellSubIDCVltM"
  High_V_Batt_Cell_V_Mtrx_1_HV1/25 -> Terminator_9/1  "HVBCVM1_CellSubIDBVltM"
  High_V_Batt_Cell_V_Mtrx_1_HV1/26 -> Terminator_10/1  "HVBCVM1_CellSubIDAVltM"
  High_V_Batt_Cell_V_Mtrx_1_HV1/27 -> Terminator_11/1  "HVBCVM1_CellSubIDAVlt"
  High_V_Batt_Cell_V_Mtrx_1_HV1/36 -> Terminator_12/1  "HVBCVM1_CellSubIDCVltV"
  High_V_Batt_Cell_V_Mtrx_1_HV1/37 -> Terminator_13/1  "HVBCVM1_CellSubIDBVltV"
  High_V_Batt_Cell_V_Mtrx_1_HV1/38 -> Terminator_14/1  "HVBCVM1_CellSubIDAVltV"
  High_V_Batt_Cell_V_Mtrx_2_HV1/1 -> Terminator_18/1  "HVBCVM2_CellOCVStat"
  High_V_Batt_Cell_V_Mtrx_2_HV1/2 -> Terminator_19/1  "HVBCVM2_CellIndx"
  High_V_Batt_Cell_V_Mtrx_2_HV1/3 -> Terminator_20/1  "HVBCVM2_CellTstSubIDCAct"
  High_V_Batt_Cell_V_Mtrx_2_HV1/4 -> Terminator_21/1  "HVBCVM2_CellTstSubIDBAct"
  High_V_Batt_Cell_V_Mtrx_2_HV1/5 -> Terminator_22/1  "HVBCVM2_CellTstSubIDAAct"
  High_V_Batt_Cell_V_Mtrx_2_HV1/6 -> Terminator_23/1  "HVBCVM2_CellSubIDCVlt"
  High_V_Batt_Cell_V_Mtrx_2_HV1/15 -> Terminator_24/1  "HVBCVM2_CellSubIDBVlt"
  High_V_Batt_Cell_V_Mtrx_2_HV1/24 -> Terminator_25/1  "HVBCVM2_CellSubIDCVltM"
  High_V_Batt_Cell_V_Mtrx_2_HV1/25 -> Terminator_26/1  "HVBCVM2_CellSubIDBVltM"
  High_V_Batt_Cell_V_Mtrx_2_HV1/26 -> Terminator_27/1  "HVBCVM2_CellSubIDAVltM"
  High_V_Batt_Cell_V_Mtrx_2_HV1/27 -> Terminator_28/1  "HVBCVM2_CellSubIDAVlt"
  High_V_Batt_Cell_V_Mtrx_2_HV1/36 -> Terminator_29/1  "HVBCVM2_CellSubIDCVltV"
  High_V_Batt_Cell_V_Mtrx_2_HV1/37 -> Terminator_30/1  "HVBCVM2_CellSubIDBVltV"
  High_V_Batt_Cell_V_Mtrx_2_HV1/38 -> Terminator_31/1  "HVBCVM2_CellSubIDAVltV"
  High_V_Batt_Cell_V_Mtrx_3_HV1/1 -> Terminator_35/1  "HVBCVM3_CellVltOCVStat"
  High_V_Batt_Cell_V_Mtrx_3_HV1/2 -> Terminator_36/1  "HVBCVM3_CellIndx"
  High_V_Batt_Cell_V_Mtrx_3_HV1/3 -> Terminator_37/1  "HVBCVM3_CellTstSubIDCAct"
  High_V_Batt_Cell_V_Mtrx_3_HV1/4 -> Terminator_38/1  "HVBCVM3_CellTstSubIDBAct"
  High_V_Batt_Cell_V_Mtrx_3_HV1/5 -> Terminator_39/1  "HVBCVM3_CellTstSubIDAAct"
  High_V_Batt_Cell_V_Mtrx_3_HV1/6 -> Terminator_40/1  "HVBCVM3_CellSubIDCVlt"
  High_V_Batt_Cell_V_Mtrx_3_HV1/15 -> Terminator_41/1  "HVBCVM3_CellSubIDBVlt"
  High_V_Batt_Cell_V_Mtrx_3_HV1/24 -> Terminator_42/1  "HVBCVM3_CellSubIDCVltM"
  High_V_Batt_Cell_V_Mtrx_3_HV1/25 -> Terminator_43/1  "HVBCVM3_CellSubIDBVltM"
  High_V_Batt_Cell_V_Mtrx_3_HV1/26 -> Terminator_44/1  "HVBCVM3_CellSubIDAVltM"
  High_V_Batt_Cell_V_Mtrx_3_HV1/27 -> Terminator_45/1  "HVBCVM3_CellSubIDAVlt"
  High_V_Batt_Cell_V_Mtrx_3_HV1/36 -> Terminator_46/1  "HVBCVM3_CellSubIDCVltV"
  High_V_Batt_Cell_V_Mtrx_3_HV1/37 -> Terminator_47/1  "HVBCVM3_CellSubIDBVltV"
  High_V_Batt_Cell_V_Mtrx_3_HV1/38 -> Terminator_48/1  "HVBCVM3_CellSubIDAVltV"
  High_V_Batt_Cell_V_Mtrx_4_HV1/1 -> Terminator_49/1  "HVBCVM4_CellVltOCVStat"
  High_V_Batt_Cell_V_Mtrx_4_HV1/2 -> Terminator_50/1  "HVBCVM4_CellIndx"
  High_V_Batt_Cell_V_Mtrx_4_HV1/3 -> Terminator_51/1  "HVBCVM4_CellTstSubIDCAct"
  High_V_Batt_Cell_V_Mtrx_4_HV1/4 -> Terminator_52/1  "HVBCVM4_CellTstSubIDBAct"
  High_V_Batt_Cell_V_Mtrx_4_HV1/5 -> Terminator_53/1  "HVBCVM4_CellTstSubIDAAct"
  High_V_Batt_Cell_V_Mtrx_4_HV1/6 -> Terminator_54/1  "HVBCVM4_CellSubIDCVlt"
  High_V_Batt_Cell_V_Mtrx_4_HV1/15 -> Terminator_55/1  "HVBCVM4_CellSubIDBVlt"
  High_V_Batt_Cell_V_Mtrx_4_HV1/24 -> Terminator_56/1  "HVBCVM4_CellSubIDCVltM"
  High_V_Batt_Cell_V_Mtrx_4_HV1/25 -> Terminator_57/1  "HVBCVM4_CellSubIDBVltM"
  High_V_Batt_Cell_V_Mtrx_4_HV1/26 -> Terminator_58/1  "HVBCVM4_CellSubIDAVltM"
  High_V_Batt_Cell_V_Mtrx_4_HV1/27 -> Terminator_59/1  "HVBCVM4_CellSubIDAVlt"
  High_V_Batt_Cell_V_Mtrx_4_HV1/36 -> Terminator_60/1  "HVBCVM4_CellSubIDCVltV"
  High_V_Batt_Cell_V_Mtrx_4_HV1/37 -> Terminator_61/1  "HVBCVM4_CellSubIDBVltV"
  High_V_Batt_Cell_V_Mtrx_4_HV1/38 -> Terminator_62/1  "HVBCVM4_CellSubIDAVltV"
  Gain5/1 -> SumCells/1, Compare To Zero5/1
  Compare To Zero5/1 -> [chsum]
  Bus Creator7/1 -> Subsystem/1(In1)
  [CellMatrixTwo] -> Bus Creator7/2
  [CellMatrixThree] -> Bus Creator7/3
  [CellMatrixFour] -> Bus Creator7/4
  [CellMatrixOne] -> Bus Creator7/1
  Subsystem/1(MinSection_PackEquivalent) -> MinSection_PackEquivalent/1
